simulink model "ForwardKinematic_YuMi"  (R2024a)
(part 8 of 23)

Jacobian_left = [(973764137223015786259973668329660771163465792108934354094153261381447822936595819206046373024901212106219886775732921677418044357043373*sin(q1L))/56784275335594288324165922491250354246378231303696723459491421810987444383859212759858675837012778559434572000489545151057390752235520000 - (89044539378776407626383878029300732391902246482356429453424426540503686155769084630894908573032444807606609378851922454344544769346221*cos(q1L))/28392137667797144162082961245625177123189115651848361729745710905493722191929606379929337918506389279717286000244772575528695376117760000 - (2436553109258773196144549622003023*cos(q6L)*((7514214926474921*cos(q5L)*(((4503599440548691*cos(q4L))/4503599627370496 - (7514214926474921*sin(q4L))/36893488147419103232)*((9007199067919185*sin(q3L)*((46370457884011341126541404977865*cos(q1L))/81129638414606681695789005144064 + (17012367886825063216155529491255*sin(q1L))/162259276829213363391578010288128))/9007199254740992 - cos(q3L)*(cos(q2L)*((1888752292310023*cos(q1L))/18014398509481984 - (5148155107303929*sin(q1L))/9007199254740992) + (7514214926474921*sin(q2L)*((5148155107303929*cos(q1L))/9007199254740992 + (1888752292310023*sin(q1L))/18014398509481984))/36893488147419103232) + (7514214926474921*sin(q3L)*((7514214926474921*cos(q2L)*((5148155107303929*cos(q1L))/9007199254740992 + (1888752292310023*sin(q1L))/18014398509481984))/36893488147419103232 - sin(q2L)*((1888752292310023*cos(q1L))/18014398509481984 - (5148155107303929*sin(q1L))/9007199254740992)))/36893488147419103232) + ((234819211581865*cos(q4L))/1152921504606846976 + (9007199067919185*sin(q4L))/9007199254740992)*((348437586779514700475067630180842053206482623665*cos(q1L))/2993155353253689176481146537402947624255349848014848 + (127834588709863499538908289888301307693646315855*sin(q1L))/5986310706507378352962293074805895248510699696029696 - (67682029681889335677290557259385*cos(q2L)*((5148155107303929*cos(q1L))/9007199254740992 + (1888752292310023*sin(q1L))/18014398509481984))/332306998946228968225951765070086144 + (9007199067919185*sin(q2L)*((1888752292310023*cos(q1L))/18014398509481984 - (5148155107303929*sin(q1L))/9007199254740992))/9007199254740992) + (7514214926474921*cos(q4L)*((9007199067919185*cos(q3L)*((46370457884011341126541404977865*cos(q1L))/81129638414606681695789005144064 + (17012367886825063216155529491255*sin(q1L))/162259276829213363391578010288128))/9007199254740992 + (7514214926474921*cos(q3L)*((7514214926474921*cos(q2L)*((5148155107303929*cos(q1L))/9007199254740992 + (1888752292310023*sin(q1L))/18014398509481984))/36893488147419103232 - sin(q2L)*((1888752292310023*cos(q1L))/18014398509481984 - (5148155107303929*sin(q1L))/9007199254740992)))/36893488147419103232 + sin(q3L)*(cos(q2L)*((1888752292310023*cos(q1L))/18014398509481984 - (5148155107303929*sin(q1L))/9007199254740992) + (7514214926474921*sin(q2L)*((5148155107303929*cos(q1L))/9007199254740992 + (1888752292310023*sin(q1L))/18014398509481984))/36893488147419103232)))/36893488147419103232))/36893488147419103232 + sin(q5L)*(((7514214926474921*cos(q4L))/36893488147419103232 + (4503599440548691*sin(q4L))/4503599627370496)*((9007199067919185*sin(q3L)*((46370457884011341126541404977865*cos(q1L))/81129638414606681695789005144064 + (17012367886825063216155529491255*sin(q1L))/162259276829213363391578010288128))/9007199254740992 - cos(q3L)*(cos(q2L)*((1888752292310023*cos(q1L))/18014398509481984 - (5148155107303929*sin(q1L))/9007199254740992) + (7514214926474921*sin(q2L)*((5148155107303929*cos(q1L))/9007199254740992 + (1888752292310023*sin(q1L))/18014398509481984))/36893488147419103232) + (7514214926474921*sin(q3L)*((7514214926474921*cos(q2L)*((5148155107303929*cos(q1L))/9007199254740992 + (1888752292310023*sin(q1L))/18014398509481984))/36893488147419103232 - sin(q2L)*((1888752292310023*cos(q1L))/18014398509481984 - (5148155107303929*sin(q1L))/9007199254740992)))/36893488147419103232) - ((9007199067919185*cos(q4L))/9007199254740992 - (234819211581865*sin(q4L))/1152921504606846976)*((348437586779514700475067630180842053206482623665*cos(q1L))/2993155353253689176481146537402947624255349848014848 + (127834588709863499538908289888301307693646315855*sin(q1L))/5986310706507378352962293074805895248510699696029696 - (67682029681889335677290557259385*cos(q2L)*((5148155107303929*cos(q1L))/9007199254740992 + (1888752292310023*sin(q1L))/18014398509481984))/332306998946228968225951765070086144 + (9007199067919185*sin(q2L)*((1888752292310023*cos(q1L))/18014398509481984 - (5148155107303929*sin(q1L))/9007199254740992))/9007199254740992) + (7514214926474921*sin(q4L)*((9007199067919185*cos(q3L)*((46370457884011341126541404977865*cos(q1L))/81129638414606681695789005144064 + (17012367886825063216155529491255*sin(q1L))/162259276829213363391578010288128))/9007199254740992 + (7514214926474921*cos(q3L)*((7514214926474921*cos(q2L)*((5148155107303929*cos(q1L))/9007199254740992 + (1888752292310023*sin(q1L))/18014398509481984))/36893488147419103232 - sin(q2L)*((1888752292310023*cos(q1L))/18014398509481984 - (5148155107303929*sin(q1L))/9007199254740992)))/36893488147419103232 + sin(q3L)*(cos(q2L)*((1888752292310023*cos(q1L))/18014398509481984 - (5148155107303929*sin(q1L))/9007199254740992) + (7514214926474921*sin(q2L)*((5148155107303929*cos(q1L))/9007199254740992 + (1888752292310023*sin(q1L))/18014398509481984))/36893488147419103232)))/36893488147419103232) - (9007199067919185*cos(q5L)*((546062636309760713610973115066597791006802105742542518556166375*cos(q1L))/113078212145816597093331040047546785012958969400039613319782796882727665664 + (200339157344278917575443724098432450908090682630030995291449625*sin(q1L))/226156424291633194186662080095093570025917938800079226639565593765455331328 - (81129635049124235038645691064225*cos(q3L)*((46370457884011341126541404977865*cos(q1L))/81129638414606681695789005144064 + (17012367886825063216155529491255*sin(q1L))/162259276829213363391578010288128))/81129638414606681695789005144064 + (2115063383689692319117831580025*sin(q3L)*((46370457884011341126541404977865*cos(q1L))/81129638414606681695789005144064 + (17012367886825063216155529491255*sin(q1L))/162259276829213363391578010288128))/10384593717069655257060992658440192 - (234819211581865*cos(q3L)*(cos(q2L)*((1888752292310023*cos(q1L))/18014398509481984 - (5148155107303929*sin(q1L))/9007199254740992) + (7514214926474921*sin(q2L)*((5148155107303929*cos(q1L))/9007199254740992 + (1888752292310023*sin(q1L))/18014398509481984))/36893488147419103232))/1152921504606846976 - (67682029681889335677290557259385*cos(q3L)*((7514214926474921*cos(q2L)*((5148155107303929*cos(q1L))/9007199254740992 + (1888752292310023*sin(q1L))/18014398509481984))/36893488147419103232 - sin(q2L)*((1888752292310023*cos(q1L))/18014398509481984 - (5148155107303929*sin(q1L))/9007199254740992)))/332306998946228968225951765070086144 - (9007199067919185*sin(q3L)*(cos(q2L)*((1888752292310023*cos(q1L))/18014398509481984 - (5148155107303929*sin(q1L))/9007199254740992) + (7514214926474921*sin(q2L)*((5148155107303929*cos(q1L))/9007199254740992 + (1888752292310023*sin(q1L))/18014398509481984))/36893488147419103232))/9007199254740992 + (1764482024691522628700660907665*sin(q3L)*((7514214926474921*cos(q2L)*((5148155107303929*cos(q1L))/9007199254740992 + (1888752292310023*sin(q1L))/18014398509481984))/36893488147419103232 - sin(q2L)*((1888752292310023*cos(q1L))/18014398509481984 - (5148155107303929*sin(q1L))/9007199254740992)))/42535295865117307932921825928971026432 - (106069577339469832923929692356850887620017617375*cos(q2L)*((5148155107303929*cos(q1L))/9007199254740992 + (1888752292310023*sin(q1L))/18014398509481984))/12554203470773361527671578846415332832204710888928069025792 + (14115856197532180673579726082375*sin(q2L)*((1888752292310023*cos(q1L))/18014398509481984 - (5148155107303929*sin(q1L))/9007199254740992))/340282366920938463463374607431768211456))/9007199254740992))/332306998946228968225951765070086144000 - (81222263116692158804177042061221826384594597321566869716687*((4503599440548691*cos(q4L))/4503599627370496 - (7514214926474921*sin(q4L))/36893488147419103232)*((9007199067919185*sin(q3L)*((46370457884011341126541404977865*cos(q1L))/81129638414606681695789005144064 + (17012367886825063216155529491255*sin(q1L))/162259276829213363391578010288128))/9007199254740992 - cos(q3L)*(cos(q2L)*((1888752292310023*cos(q1L))/18014398509481984 - (5148155107303929*sin(q1L))/9007199254740992) + (7514214926474921*sin(q2L)*((5148155107303929*cos(q1L))/9007199254740992 + (1888752292310023*sin(q1L))/18014398509481984))/36893488147419103232) + (7514214926474921*sin(q3L)*((7514214926474921*cos(q2L)*((5148155107303929*cos(q1L))/9007199254740992 + (1888752292310023*sin(q1L))/18014398509481984))/36893488147419103232 - sin(q2L)*((1888752292310023*cos(q1L))/18014398509481984 - (5148155107303929*sin(q1L))/9007199254740992)))/36893488147419103232))/306499108173177771671669405430061836723747824436720435200000 - (81*((7514214926474921*cos(q4L))/36893488147419103232 + (4503599440548691*sin(q4L))/4503599627370496)*((9007199067919185*sin(q3L)*((46370457884011341126541404977865*cos(q1L))/81129638414606681695789005144064 + (17012367886825063216155529491255*sin(q1L))/162259276829213363391578010288128))/9007199254740992 - cos(q3L)*(cos(q2L)*((1888752292310023*cos(q1L))/18014398509481984 - (5148155107303929*sin(q1L))/9007199254740992) + (7514214926474921*sin(q2L)*((5148155107303929*cos(q1L))/9007199254740992 + (1888752292310023*sin(q1L))/18014398509481984))/36893488147419103232) + (7514214926474921*sin(q3L)*((7514214926474921*cos(q2L)*((5148155107303929*cos(q1L))/9007199254740992 + (1888752292310023*sin(q1L))/18014398509481984))/36893488147419103232 - sin(q2L)*((1888752292310023*cos(q1L))/18014398509481984 - (5148155107303929*sin(q1L))/9007199254740992)))/36893488147419103232))/2000 - (27*cos(q6L)*(cos(q5L)*(((7514214926474921*cos(q4L))/36893488147419103232 + (4503599440548691*sin(q4L))/4503599627370496)*((9007199067919185*sin(q3L)*((46370457884011341126541404977865*cos(q1L))/81129638414606681695789005144064 + (17012367886825063216155529491255*sin(q1L))/162259276829213363391578010288128))/9007199254740992 - cos(q3L)*(cos(q2L)*((1888752292310023*cos(q1L))/18014398509481984 - (5148155107303929*sin(q1L))/9007199254740992) + (7514214926474921*sin(q2L)*((5148155107303929*cos(q1L))/9007199254740992 + (1888752292310023*sin(q1L))/18014398509481984))/36893488147419103232) + (7514214926474921*sin(q3L)*((7514214926474921*cos(q2L)*((5148155107303929*cos(q1L))/9007199254740992 + (1888752292310023*sin(q1L))/18014398509481984))/36893488147419103232 - sin(q2L)*((1888752292310023*cos(q1L))/18014398509481984 - (5148155107303929*sin(q1L))/9007199254740992)))/36893488147419103232) - ((9007199067919185*cos(q4L))/9007199254740992 - (234819211581865*sin(q4L))/1152921504606846976)*((348437586779514700475067630180842053206482623665*cos(q1L))/2993155353253689176481146537402947624255349848014848 + (127834588709863499538908289888301307693646315855*sin(q1L))/5986310706507378352962293074805895248510699696029696 - (67682029681889335677290557259385*cos(q2L)*((5148155107303929*cos(q1L))/9007199254740992 + (1888752292310023*sin(q1L))/18014398509481984))/332306998946228968225951765070086144 + (9007199067919185*sin(q2L)*((1888752292310023*cos(q1L))/18014398509481984 - (5148155107303929*sin(q1L))/9007199254740992))/9007199254740992) + (7514214926474921*sin(q4L)*((9007199067919185*cos(q3L)*((46370457884011341126541404977865*cos(q1L))/81129638414606681695789005144064 + (17012367886825063216155529491255*sin(q1L))/162259276829213363391578010288128))/9007199254740992 + (7514214926474921*cos(q3L)*((7514214926474921*cos(q2L)*((5148155107303929*cos(q1L))/9007199254740992 + (1888752292310023*sin(q1L))/18014398509481984))/36893488147419103232 - sin(q2L)*((1888752292310023*cos(q1L))/18014398509481984 - (5148155107303929*sin(q1L))/9007199254740992)))/36893488147419103232 + sin(q3L)*(cos(q2L)*((1888752292310023*cos(q1L))/18014398509481984 - (5148155107303929*sin(q1L))/9007199254740992) + (7514214926474921*sin(q2L)*((5148155107303929*cos(q1L))/9007199254740992 + (1888752292310023*sin(q1L))/18014398509481984))/36893488147419103232)))/36893488147419103232) - (7514214926474921*sin(q5L)*(((4503599440548691*cos(q4L))/4503599627370496 - (7514214926474921*sin(q4L))/36893488147419103232)*((9007199067919185*sin(q3L)*((46370457884011341126541404977865*cos(q1L))/81129638414606681695789005144064 + (17012367886825063216155529491255*sin(q1L))/162259276829213363391578010288128))/9007199254740992 - cos(q3L)*(cos(q2L)*((1888752292310023*cos(q1L))/18014398509481984 - (5148155107303929*sin(q1L))/9007199254740992) + (7514214926474921*sin(q2L)*((5148155107303929*cos(q1L))/9007199254740992 + (1888752292310023*sin(q1L))/18014398509481984))/36893488147419103232) + (7514214926474921*sin(q3L)*((7514214926474921*cos(q2L)*((5148155107303929*cos(q1L))/9007199254740992 + (1888752292310023*sin(q1L))/18014398509481984))/36893488147419103232 - sin(q2L)*((1888752292310023*cos(q1L))/18014398509481984 - (5148155107303929*sin(q1L))/9007199254740992)))/36893488147419103232) + ((234819211581865*cos(q4L))/1152921504606846976 + (9007199067919185*sin(q4L))/9007199254740992)*((348437586779514700475067630180842053206482623665*cos(q1L))/2993155353253689176481146537402947624255349848014848 + (127834588709863499538908289888301307693646315855*sin(q1L))/5986310706507378352962293074805895248510699696029696 - (67682029681889335677290557259385*cos(q2L)*((5148155107303929*cos(q1L))/9007199254740992 + (1888752292310023*sin(q1L))/18014398509481984))/332306998946228968225951765070086144 + (9007199067919185*sin(q2L)*((1888752292310023*cos(q1L))/18014398509481984 - (5148155107303929*sin(q1L))/9007199254740992))/9007199254740992) + (7514214926474921*cos(q4L)*((9007199067919185*cos(q3L)*((46370457884011341126541404977865*cos(q1L))/81129638414606681695789005144064 + (17012367886825063216155529491255*sin(q1L))/162259276829213363391578010288128))/9007199254740992 + (7514214926474921*cos(q3L)*((7514214926474921*cos(q2L)*((5148155107303929*cos(q1L))/9007199254740992 + (1888752292310023*sin(q1L))/18014398509481984))/36893488147419103232 - sin(q2L)*((1888752292310023*cos(q1L))/18014398509481984 - (5148155107303929*sin(q1L))/9007199254740992)))/36893488147419103232 + sin(q3L)*(cos(q2L)*((1888752292310023*cos(q1L))/18014398509481984 - (5148155107303929*sin(q1L))/9007199254740992) + (7514214926474921*sin(q2L)*((5148155107303929*cos(q1L))/9007199254740992 + (1888752292310023*sin(q1L))/18014398509481984))/36893488147419103232)))/36893488147419103232))/36893488147419103232 + (9007199067919185*sin(q5L)*((546062636309760713610973115066597791006802105742542518556166375*cos(q1L))/113078212145816597093331040047546785012958969400039613319782796882727665664 + (200339157344278917575443724098432450908090682630030995291449625*sin(q1L))/226156424291633194186662080095093570025917938800079226639565593765455331328 - (81129635049124235038645691064225*cos(q3L)*((46370457884011341126541404977865*cos(q1L))/81129638414606681695789005144064 + (17012367886825063216155529491255*sin(q1L))/162259276829213363391578010288128))/81129638414606681695789005144064 + (2115063383689692319117831580025*sin(q3L)*((46370457884011341126541404977865*cos(q1L))/81129638414606681695789005144064 + (17012367886825063216155529491255*sin(q1L))/162259276829213363391578010288128))/10384593717069655257060992658440192 - (234819211581865*cos(q3L)*(cos(q2L)*((1888752292310023*cos(q1L))/18014398509481984 - (5148155107303929*sin(q1L))/9007199254740992) + (7514214926474921*sin(q2L)*((5148155107303929*cos(q1L))/9007199254740992 + (1888752292310023*sin(q1L))/18014398509481984))/36893488147419103232))/1152921504606846976 - (67682029681889335677290557259385*cos(q3L)*((7514214926474921*cos(q2L)*((5148155107303929*cos(q1L))/9007199254740992 + (1888752292310023*sin(q1L))/18014398509481984))/36893488147419103232 - sin(q2L)*((1888752292310023*cos(q1L))/18014398509481984 - (5148155107303929*sin(q1L))/9007199254740992)))/332306998946228968225951765070086144 - (9007199067919185*sin(q3L)*(cos(q2L)*((1888752292310023*cos(q1L))/18014398509481984 - (5148155107303929*sin(q1L))/9007199254740992) + (7514214926474921*sin(q2L)*((5148155107303929*cos(q1L))/9007199254740992 + (1888752292310023*sin(q1L))/18014398509481984))/36893488147419103232))/9007199254740992 + (1764482024691522628700660907665*sin(q3L)*((7514214926474921*cos(q2L)*((5148155107303929*cos(q1L))/9007199254740992 + (1888752292310023*sin(q1L))/18014398509481984))/36893488147419103232 - sin(q2L)*((1888752292310023*cos(q1L))/18014398509481984 - (5148155107303929*sin(q1L))/9007199254740992)))/42535295865117307932921825928971026432 - (106069577339469832923929692356850887620017617375*cos(q2L)*((5148155107303929*cos(q1L))/9007199254740992 + (1888752292310023*sin(q1L))/18014398509481984))/12554203470773361527671578846415332832204710888928069025792 + (14115856197532180673579726082375*sin(q2L)*((1888752292310023*cos(q1L))/18014398509481984 - (5148155107303929*sin(q1L))/9007199254740992))/340282366920938463463374607431768211456))/9007199254740992))/1000 - (202883803014822867*sin(q6L)*((7514214926474921*cos(q5L)*(((4503599440548691*cos(q4L))/4503599627370496 - (7514214926474921*sin(q4L))/36893488147419103232)*((9007199067919185*sin(q3L)*((46370457884011341126541404977865*cos(q1L))/81129638414606681695789005144064 + (17012367886825063216155529491255*sin(q1L))/162259276829213363391578010288128))/9007199254740992 - cos(q3L)*(cos(q2L)*((1888752292310023*cos(q1L))/18014398509481984 - (5148155107303929*sin(q1L))/9007199254740992) + (7514214926474921*sin(q2L)*((5148155107303929*cos(q1L))/9007199254740992 + (1888752292310023*sin(q1L))/18014398509481984))/36893488147419103232) + (7514214926474921*sin(q3L)*((7514214926474921*cos(q2L)*((5148155107303929*cos(q1L))/9007199254740992 + (1888752292310023*sin(q1L))/18014398509481984))/36893488147419103232 - sin(q2L)*((1888752292310023*cos(q1L))/18014398509481984 - (5148155107303929*sin(q1L))/9007199254740992)))/36893488147419103232) + ((234819211581865*cos(q4L))/1152921504606846976 + (9007199067919185*sin(q4L))/9007199254740992)*((348437586779514700475067630180842053206482623665*cos(q1L))/2993155353253689176481146537402947624255349848014848 + (127834588709863499538908289888301307693646315855*sin(q1L))/5986310706507378352962293074805895248510699696029696 - (67682029681889335677290557259385*cos(q2L)*((5148155107303929*cos(q1L))/9007199254740992 + (1888752292310023*sin(q1L))/18014398509481984))/332306998946228968225951765070086144 + (9007199067919185*sin(q2L)*((1888752292310023*cos(q1L))/18014398509481984 - (5148155107303929*sin(q1L))/9007199254740992))/9007199254740992) + (7514214926474921*cos(q4L)*((9007199067919185*cos(q3L)*((46370457884011341126541404977865*cos(q1L))/81129638414606681695789005144064 + (17012367886825063216155529491255*sin(q1L))/162259276829213363391578010288128))/9007199254740992 + (7514214926474921*cos(q3L)*((7514214926474921*cos(q2L)*((5148155107303929*cos(q1L))/9007199254740992 + (1888752292310023*sin(q1L))/18014398509481984))/36893488147419103232 - sin(q2L)*((1888752292310023*cos(q1L))/18014398509481984 - (5148155107303929*sin(q1L))/9007199254740992)))/36893488147419103232 + sin(q3L)*(cos(q2L)*((1888752292310023*cos(q1L))/18014398509481984 - (5148155107303929*sin(q1L))/9007199254740992) + (7514214926474921*sin(q2L)*((5148155107303929*cos(q1L))/9007199254740992 + (1888752292310023*sin(q1L))/18014398509481984))/36893488147419103232)))/36893488147419103232))/36893488147419103232 + sin(q5L)*(((7514214926474921*cos(q4L))/36893488147419103232 + (4503599440548691*sin(q4L))/4503599627370496)*((9007199067919185*sin(q3L)*((46370457884011341126541404977865*cos(q1L))/81129638414606681695789005144064 + (17012367886825063216155529491255*sin(q1L))/162259276829213363391578010288128))/9007199254740992 - cos(q3L)*(cos(q2L)*((1888752292310023*cos(q1L))/18014398509481984 - (5148155107303929*sin(q1L))/9007199254740992) + (7514214926474921*sin(q2L)*((5148155107303929*cos(q1L))/9007199254740992 + (1888752292310023*sin(q1L))/18014398509481984))/36893488147419103232) + (7514214926474921*sin(q3L)*((7514214926474921*cos(q2L)*((5148155107303929*cos(q1L))/9007199254740992 + (1888752292310023*sin(q1L))/18014398509481984))/36893488147419103232 - sin(q2L)*((1888752292310023*cos(q1L))/18014398509481984 - (5148155107303929*sin(q1L))/9007199254740992)))/36893488147419103232) - ((9007199067919185*cos(q4L))/9007199254740992 - (234819211581865*sin(q4L))/1152921504606846976)*((348437586779514700475067630180842053206482623665*cos(q1L))/2993155353253689176481146537402947624255349848014848 + (127834588709863499538908289888301307693646315855*sin(q1L))/5986310706507378352962293074805895248510699696029696 - (67682029681889335677290557259385*cos(q2L)*((5148155107303929*cos(q1L))/9007199254740992 + (1888752292310023*sin(q1L))/18014398509481984))/332306998946228968225951765070086144 + (9007199067919185*sin(q2L)*((1888752292310023*cos(q1L))/18014398509481984 - (5148155107303929*sin(q1L))/9007199254740992))/9007199254740992) + (7514214926474921*sin(q4L)*((9007199067919185*cos(q3L)*((46370457884011341126541404977865*cos(q1L))/81129638414606681695789005144064 + (17012367886825063216155529491255*sin(q1L))/162259276829213363391578010288128))/9007199254740992 + (7514214926474921*cos(q3L)*((7514214926474921*cos(q2L)*((5148155107303929*cos(q1L))/9007199254740992 + (1888752292310023*sin(q1L))/18014398509481984))/36893488147419103232 - sin(q2L)*((1888752292310023*cos(q1L))/18014398509481984 - (5148155107303929*sin(q1L))/9007199254740992)))/36893488147419103232 + sin(q3L)*(cos(q2L)*((1888752292310023*cos(q1L))/18014398509481984 - (5148155107303929*sin(q1L))/9007199254740992) + (7514214926474921*sin(q2L)*((5148155107303929*cos(q1L))/9007199254740992 + (1888752292310023*sin(q1L))/18014398509481984))/36893488147419103232)))/36893488147419103232) - (9007199067919185*cos(q5L)*((546062636309760713610973115066597791006802105742542518556166375*cos(q1L))/113078212145816597093331040047546785012958969400039613319782796882727665664 + (200339157344278917575443724098432450908090682630030995291449625*sin(q1L))/226156424291633194186662080095093570025917938800079226639565593765455331328 - (81129635049124235038645691064225*cos(q3L)*((46370457884011341126541404977865*cos(q1L))/81129638414606681695789005144064 + (17012367886825063216155529491255*sin(q1L))/162259276829213363391578010288128))/81129638414606681695789005144064 + (2115063383689692319117831580025*sin(q3L)*((46370457884011341126541404977865*cos(q1L))/81129638414606681695789005144064 + (17012367886825063216155529491255*sin(q1L))/162259276829213363391578010288128))/10384593717069655257060992658440192 - (234819211581865*cos(q3L)*(cos(q2L)*((1888752292310023*cos(q1L))/18014398509481984 - (5148155107303929*sin(q1L))/9007199254740992) + (7514214926474921*sin(q2L)*((5148155107303929*cos(q1L))/9007199254740992 + (1888752292310023*sin(q1L))/18014398509481984))/36893488147419103232))/1152921504606846976 - (67682029681889335677290557259385*cos(q3L)*((7514214926474921*cos(q2L)*((5148155107303929*cos(q1L))/9007199254740992 + (1888752292310023*sin(q1L))/18014398509481984))/36893488147419103232 - sin(q2L)*((1888752292310023*cos(q1L))/18014398509481984 - (5148155107303929*sin(q1L))/9007199254740992)))/332306998946228968225951765070086144 - (9007199067919185*sin(q3L)*(cos(q2L)*((1888752292310023*cos(q1L))/18014398509481984 - (5148155107303929*sin(q1L))/9007199254740992) + (7514214926474921*sin(q2L)*((5148155107303929*cos(q1L))/9007199254740992 + (1888752292310023*sin(q1L))/18014398509481984))/36893488147419103232))/9007199254740992 + (1764482024691522628700660907665*sin(q3L)*((7514214926474921*cos(q2L)*((5148155107303929*cos(q1L))/9007199254740992 + (1888752292310023*sin(q1L))/18014398509481984))/36893488147419103232 - sin(q2L)*((1888752292310023*cos(q1L))/18014398509481984 - (5148155107303929*sin(q1L))/9007199254740992)))/42535295865117307932921825928971026432 - (106069577339469832923929692356850887620017617375*cos(q2L)*((5148155107303929*cos(q1L))/9007199254740992 + (1888752292310023*sin(q1L))/18014398509481984))/12554203470773361527671578846415332832204710888928069025792 + (14115856197532180673579726082375*sin(q2L)*((1888752292310023*cos(q1L))/18014398509481984 - (5148155107303929*sin(q1L))/9007199254740992))/340282366920938463463374607431768211456))/9007199254740992))/36893488147419103232000 + (324259171862923063*sin(q6L)*(cos(q5L)*(((7514214926474921*cos(q4L))/36893488147419103232 + (4503599440548691*sin(q4L))/4503599627370496)*((9007199067919185*sin(q3L)*((46370457884011341126541404977865*cos(q1L))/81129638414606681695789005144064 + (17012367886825063216155529491255*sin(q1L))/162259276829213363391578010288128))/9007199254740992 - cos(q3L)*(cos(q2L)*((1888752292310023*cos(q1L))/18014398509481984 - (5148155107303929*sin(q1L))/9007199254740992) + (7514214926474921*sin(q2L)*((5148155107303929*cos(q1L))/9007199254740992 + (1888752292310023*sin(q1L))/18014398509481984))/36893488147419103232) + (7514214926474921*sin(q3L)*((7514214926474921*cos(q2L)*((5148155107303929*cos(q1L))/9007199254740992 + (1888752292310023*sin(q1L))/18014398509481984))/36893488147419103232 - sin(q2L)*((1888752292310023*cos(q1L))/18014398509481984 - (5148155107303929*sin(q1L))/9007199254740992)))/36893488147419103232) - ((9007199067919185*cos(q4L))/9007199254740992 - (234819211581865*sin(q4L))/1152921504606846976)*((348437586779514700475067630180842053206482623665*cos(q1L))/2993155353253689176481146537402947624255349848014848 + (127834588709863499538908289888301307693646315855*sin(q1L))/5986310706507378352962293074805895248510699696029696 - (67682029681889335677290557259385*cos(q2L)*((5148155107303929*cos(q1L))/9007199254740992 + (1888752292310023*sin(q1L))/18014398509481984))/332306998946228968225951765070086144 + (9007199067919185*sin(q2L)*((1888752292310023*cos(q1L))/18014398509481984 - (5148155107303929*sin(q1L))/9007199254740992))/9007199254740992) + (7514214926474921*sin(q4L)*((9007199067919185*cos(q3L)*((46370457884011341126541404977865*cos(q1L))/81129638414606681695789005144064 + (17012367886825063216155529491255*sin(q1L))/162259276829213363391578010288128))/9007199254740992 + (7514214926474921*cos(q3L)*((7514214926474921*cos(q2L)*((5148155107303929*cos(q1L))/9007199254740992 + (1888752292310023*sin(q1L))/18014398509481984))/36893488147419103232 - sin(q2L)*((1888752292310023*cos(q1L))/18014398509481984 - (5148155107303929*sin(q1L))/9007199254740992)))/36893488147419103232 + sin(q3L)*(cos(q2L)*((1888752292310023*cos(q1L))/18014398509481984 - (5148155107303929*sin(q1L))/9007199254740992) + (7514214926474921*sin(q2L)*((5148155107303929*cos(q1L))/9007199254740992 + (1888752292310023*sin(q1L))/18014398509481984))/36893488147419103232)))/36893488147419103232) - (7514214926474921*sin(q5L)*(((4503599440548691*cos(q4L))/4503599627370496 - (7514214926474921*sin(q4L))/36893488147419103232)*((9007199067919185*sin(q3L)*((46370457884011341126541404977865*cos(q1L))/81129638414606681695789005144064 + (17012367886825063216155529491255*sin(q1L))/162259276829213363391578010288128))/9007199254740992 - cos(q3L)*(cos(q2L)*((1888752292310023*cos(q1L))/18014398509481984 - (5148155107303929*sin(q1L))/9007199254740992) + (7514214926474921*sin(q2L)*((5148155107303929*cos(q1L))/9007199254740992 + (1888752292310023*sin(q1L))/18014398509481984))/36893488147419103232) + (7514214926474921*sin(q3L)*((7514214926474921*cos(q2L)*((5148155107303929*cos(q1L))/9007199254740992 + (1888752292310023*sin(q1L))/18014398509481984))/36893488147419103232 - sin(q2L)*((1888752292310023*cos(q1L))/18014398509481984 - (5148155107303929*sin(q1L))/9007199254740992)))/36893488147419103232) + ((234819211581865*cos(q4L))/1152921504606846976 + (9007199067919185*sin(q4L))/9007199254740992)*((348437586779514700475067630180842053206482623665*cos(q1L))/2993155353253689176481146537402947624255349848014848 + (127834588709863499538908289888301307693646315855*sin(q1L))/5986310706507378352962293074805895248510699696029696 - (67682029681889335677290557259385*cos(q2L)*((5148155107303929*cos(q1L))/9007199254740992 + (1888752292310023*sin(q1L))/18014398509481984))/332306998946228968225951765070086144 + (9007199067919185*sin(q2L)*((1888752292310023*cos(q1L))/18014398509481984 - (5148155107303929*sin(q1L))/9007199254740992))/9007199254740992) + (7514214926474921*cos(q4L)*((9007199067919185*cos(q3L)*((46370457884011341126541404977865*cos(q1L))/81129638414606681695789005144064 + (17012367886825063216155529491255*sin(q1L))/162259276829213363391578010288128))/9007199254740992 + (7514214926474921*cos(q3L)*((7514214926474921*cos(q2L)*((5148155107303929*cos(q1L))/9007199254740992 + (1888752292310023*sin(q1L))/18014398509481984))/36893488147419103232 - sin(q2L)*((1888752292310023*cos(q1L))/18014398509481984 - (5148155107303929*sin(q1L))/9007199254740992)))/36893488147419103232 + sin(q3L)*(cos(q2L)*((1888752292310023*cos(q1L))/18014398509481984 - (5148155107303929*sin(q1L))/9007199254740992) + (7514214926474921*sin(q2L)*((5148155107303929*cos(q1L))/9007199254740992 + (1888752292310023*sin(q1L))/18014398509481984))/36893488147419103232)))/36893488147419103232))/36893488147419103232 + (9007199067919185*sin(q5L)*((546062636309760713610973115066597791006802105742542518556166375*cos(q1L))/113078212145816597093331040047546785012958969400039613319782796882727665664 + (200339157344278917575443724098432450908090682630030995291449625*sin(q1L))/226156424291633194186662080095093570025917938800079226639565593765455331328 - (81129635049124235038645691064225*cos(q3L)*((46370457884011341126541404977865*cos(q1L))/81129638414606681695789005144064 + (17012367886825063216155529491255*sin(q1L))/162259276829213363391578010288128))/81129638414606681695789005144064 + (2115063383689692319117831580025*sin(q3L)*((46370457884011341126541404977865*cos(q1L))/81129638414606681695789005144064 + (17012367886825063216155529491255*sin(q1L))/162259276829213363391578010288128))/10384593717069655257060992658440192 - (234819211581865*cos(q3L)*(cos(q2L)*((1888752292310023*cos(q1L))/18014398509481984 - (5148155107303929*sin(q1L))/9007199254740992) + (7514214926474921*sin(q2L)*((5148155107303929*cos(q1L))/9007199254740992 + (1888752292310023*sin(q1L))/18014398509481984))/36893488147419103232))/1152921504606846976 - (67682029681889335677290557259385*cos(q3L)*((7514214926474921*cos(q2L)*((5148155107303929*cos(q1L))/9007199254740992 + (1888752292310023*sin(q1L))/18014398509481984))/36893488147419103232 - sin(q2L)*((1888752292310023*cos(q1L))/18014398509481984 - (5148155107303929*sin(q1L))/9007199254740992)))/332306998946228968225951765070086144 - (9007199067919185*sin(q3L)*(cos(q2L)*((1888752292310023*cos(q1L))/18014398509481984 - (5148155107303929*sin(q1L))/9007199254740992) + (7514214926474921*sin(q2L)*((5148155107303929*cos(q1L))/9007199254740992 + (1888752292310023*sin(q1L))/18014398509481984))/36893488147419103232))/9007199254740992 + (1764482024691522628700660907665*sin(q3L)*((7514214926474921*cos(q2L)*((5148155107303929*cos(q1L))/9007199254740992 + (1888752292310023*sin(q1L))/18014398509481984))/36893488147419103232 - sin(q2L)*((1888752292310023*cos(q1L))/18014398509481984 - (5148155107303929*sin(q1L))/9007199254740992)))/42535295865117307932921825928971026432 - (106069577339469832923929692356850887620017617375*cos(q2L)*((5148155107303929*cos(q1L))/9007199254740992 + (1888752292310023*sin(q1L))/18014398509481984))/12554203470773361527671578846415332832204710888928069025792 + (14115856197532180673579726082375*sin(q2L)*((1888752292310023*cos(q1L))/18014398509481984 - (5148155107303929*sin(q1L))/9007199254740992))/340282366920938463463374607431768211456))/9007199254740992))/9007199254740992000 + (83301539375654672537075965313343183841442266989297270401707771044036658496661398777306991*cos(q3L)*((46370457884011341126541404977865*cos(q1L))/81129638414606681695789005144064 + (17012367886825063216155529491255*sin(q1L))/162259276829213363391578010288128))/4074071952668972172536891376818756322102936787331872501272280898708762599526673412366794752000 - (109198173955282063961996941994332957526645881091499469714283881779231664456243735535448036415347*sin(q3L)*((46370457884011341126541404977865*cos(q1L))/81129638414606681695789005144064 + (17012367886825063216155529491255*sin(q1L))/162259276829213363391578010288128))/2607406049708142190423610481164004046145879543892398400814259775173608063697070983914748641280000 + (81*((9007199067919185*cos(q4L))/9007199254740992 - (234819211581865*sin(q4L))/1152921504606846976)*((348437586779514700475067630180842053206482623665*cos(q1L))/2993155353253689176481146537402947624255349848014848 + (127834588709863499538908289888301307693646315855*sin(q1L))/5986310706507378352962293074805895248510699696029696 - (67682029681889335677290557259385*cos(q2L)*((5148155107303929*cos(q1L))/9007199254740992 + (1888752292310023*sin(q1L))/18014398509481984))/332306998946228968225951765070086144 + (9007199067919185*sin(q2L)*((1888752292310023*cos(q1L))/18014398509481984 - (5148155107303929*sin(q1L))/9007199254740992))/9007199254740992))/2000 - (81222263116692158804177042061221826384594597321566869716687*((234819211581865*cos(q4L))/1152921504606846976 + (9007199067919185*sin(q4L))/9007199254740992)*((348437586779514700475067630180842053206482623665*cos(q1L))/2993155353253689176481146537402947624255349848014848 + (127834588709863499538908289888301307693646315855*sin(q1L))/5986310706507378352962293074805895248510699696029696 - (67682029681889335677290557259385*cos(q2L)*((5148155107303929*cos(q1L))/9007199254740992 + (1888752292310023*sin(q1L))/18014398509481984))/332306998946228968225951765070086144 + (9007199067919185*sin(q2L)*((1888752292310023*cos(q1L))/18014398509481984 - (5148155107303929*sin(q1L))/9007199254740992))/9007199254740992))/306499108173177771671669405430061836723747824436720435200000 + (60617164743372705924380750591060836759586313939367162716784907429017787816377231*cos(q3L)*(cos(q2L)*((1888752292310023*cos(q1L))/18014398509481984 - (5148155107303929*sin(q1L))/9007199254740992) + (7514214926474921*sin(q2L)*((5148155107303929*cos(q1L))/9007199254740992 + (1888752292310023*sin(q1L))/18014398509481984))/36893488147419103232))/1447401115466452442794637312608598848165874808320507050493219800098914120499200000 + (347469655025336708709976918716104493695816557877713443586884917071777956519687017125887603*cos(q3L)*((7514214926474921*cos(q2L)*((5148155107303929*cos(q1L))/9007199254740992 + (1888752292310023*sin(q1L))/18014398509481984))/36893488147419103232 - sin(q2L)*((1888752292310023*cos(q1L))/18014398509481984 - (5148155107303929*sin(q1L))/9007199254740992)))/83436993590660550093555535397248129476668145404556748826056312805555458038306271485271956520960000 + (712008244765680093343103025701132101054572137019*cos(q5L)*(((4503599440548691*cos(q4L))/4503599627370496 - (7514214926474921*sin(q4L))/36893488147419103232)*((9007199067919185*sin(q3L)*((46370457884011341126541404977865*cos(q1L))/81129638414606681695789005144064 + (17012367886825063216155529491255*sin(q1L))/162259276829213363391578010288128))/9007199254740992 - cos(q3L)*(cos(q2L)*((1888752292310023*cos(q1L))/18014398509481984 - (5148155107303929*sin(q1L))/9007199254740992) + (7514214926474921*sin(q2L)*((5148155107303929*cos(q1L))/9007199254740992 + (1888752292310023*sin(q1L))/18014398509481984))/36893488147419103232) + (7514214926474921*sin(q3L)*((7514214926474921*cos(q2L)*((5148155107303929*cos(q1L))/9007199254740992 + (1888752292310023*sin(q1L))/18014398509481984))/36893488147419103232 - sin(q2L)*((1888752292310023*cos(q1L))/18014398509481984 - (5148155107303929*sin(q1L))/9007199254740992)))/36893488147419103232) + ((234819211581865*cos(q4L))/1152921504606846976 + (9007199067919185*sin(q4L))/9007199254740992)*((348437586779514700475067630180842053206482623665*cos(q1L))/2993155353253689176481146537402947624255349848014848 + (127834588709863499538908289888301307693646315855*sin(q1L))/5986310706507378352962293074805895248510699696029696 - (67682029681889335677290557259385*cos(q2L)*((5148155107303929*cos(q1L))/9007199254740992 + (1888752292310023*sin(q1L))/18014398509481984))/332306998946228968225951765070086144 + (9007199067919185*sin(q2L)*((1888752292310023*cos(q1L))/18014398509481984 - (5148155107303929*sin(q1L))/9007199254740992))/9007199254740992) + (7514214926474921*cos(q4L)*((9007199067919185*cos(q3L)*((46370457884011341126541404977865*cos(q1L))/81129638414606681695789005144064 + (17012367886825063216155529491255*sin(q1L))/162259276829213363391578010288128))/9007199254740992 + (7514214926474921*cos(q3L)*((7514214926474921*cos(q2L)*((5148155107303929*cos(q1L))/9007199254740992 + (1888752292310023*sin(q1L))/18014398509481984))/36893488147419103232 - sin(q2L)*((1888752292310023*cos(q1L))/18014398509481984 - (5148155107303929*sin(q1L))/9007199254740992)))/36893488147419103232 + sin(q3L)*(cos(q2L)*((1888752292310023*cos(q1L))/18014398509481984 - (5148155107303929*sin(q1L))/9007199254740992) + (7514214926474921*sin(q2L)*((5148155107303929*cos(q1L))/9007199254740992 + (1888752292310023*sin(q1L))/18014398509481984))/36893488147419103232)))/36893488147419103232))/2451992865385422173373355243440494693789982595493763481600 + (46241644459901303158631016767207157814229090534989303509431886332469146043*sin(q3L)*(cos(q2L)*((1888752292310023*cos(q1L))/18014398509481984 - (5148155107303929*sin(q1L))/9007199254740992) + (7514214926474921*sin(q2L)*((5148155107303929*cos(q1L))/9007199254740992 + (1888752292310023*sin(q1L))/18014398509481984))/36893488147419103232))/2261564242916331941866620800950935700259179388000792266395655937654553313280000 - (455490404115240510935077772268745492204390157443214084883134054419271951750419293234291596923751*sin(q3L)*((7514214926474921*cos(q2L)*((5148155107303929*cos(q1L))/9007199254740992 + (1888752292310023*sin(q1L))/18014398509481984))/36893488147419103232 - sin(q2L)*((1888752292310023*cos(q1L))/18014398509481984 - (5148155107303929*sin(q1L))/9007199254740992)))/53399675898022752059875542654238802865067613058916319248676040195555493144516013750574052173414400000 - (202883803014822867*sin(q5L)*(((4503599440548691*cos(q4L))/4503599627370496 - (7514214926474921*sin(q4L))/36893488147419103232)*((9007199067919185*sin(q3L)*((46370457884011341126541404977865*cos(q1L))/81129638414606681695789005144064 + (17012367886825063216155529491255*sin(q1L))/162259276829213363391578010288128))/9007199254740992 - cos(q3L)*(cos(q2L)*((1888752292310023*cos(q1L))/18014398509481984 - (5148155107303929*sin(q1L))/9007199254740992) + (7514214926474921*sin(q2L)*((5148155107303929*cos(q1L))/9007199254740992 + (1888752292310023*sin(q1L))/18014398509481984))/36893488147419103232) + (7514214926474921*sin(q3L)*((7514214926474921*cos(q2L)*((5148155107303929*cos(q1L))/9007199254740992 + (1888752292310023*sin(q1L))/18014398509481984))/36893488147419103232 - sin(q2L)*((1888752292310023*cos(q1L))/18014398509481984 - (5148155107303929*sin(q1L))/9007199254740992)))/36893488147419103232) + ((234819211581865*cos(q4L))/1152921504606846976 + (9007199067919185*sin(q4L))/9007199254740992)*((348437586779514700475067630180842053206482623665*cos(q1L))/2993155353253689176481146537402947624255349848014848 + (127834588709863499538908289888301307693646315855*sin(q1L))/5986310706507378352962293074805895248510699696029696 - (67682029681889335677290557259385*cos(q2L)*((5148155107303929*cos(q1L))/9007199254740992 + (1888752292310023*sin(q1L))/18014398509481984))/332306998946228968225951765070086144 + (9007199067919185*sin(q2L)*((1888752292310023*cos(q1L))/18014398509481984 - (5148155107303929*sin(q1L))/9007199254740992))/9007199254740992) + (7514214926474921*cos(q4L)*((9007199067919185*cos(q3L)*((46370457884011341126541404977865*cos(q1L))/81129638414606681695789005144064 + (17012367886825063216155529491255*sin(q1L))/162259276829213363391578010288128))/9007199254740992 + (7514214926474921*cos(q3L)*((7514214926474921*cos(q2L)*((5148155107303929*cos(q1L))/9007199254740992 + (1888752292310023*sin(q1L))/18014398509481984))/36893488147419103232 - sin(q2L)*((1888752292310023*cos(q1L))/18014398509481984 - (5148155107303929*sin(q1L))/9007199254740992)))/36893488147419103232 + sin(q3L)*(cos(q2L)*((1888752292310023*cos(q1L))/18014398509481984 - (5148155107303929*sin(q1L))/9007199254740992) + (7514214926474921*sin(q2L)*((5148155107303929*cos(q1L))/9007199254740992 + (1888752292310023*sin(q1L))/18014398509481984))/36893488147419103232)))/36893488147419103232))/36893488147419103232000 + (27*cos(q5L)*(((7514214926474921*cos(q4L))/36893488147419103232 + (4503599440548691*sin(q4L))/4503599627370496)*((9007199067919185*sin(q3L)*((46370457884011341126541404977865*cos(q1L))/81129638414606681695789005144064 + (17012367886825063216155529491255*sin(q1L))/162259276829213363391578010288128))/9007199254740992 - cos(q3L)*(cos(q2L)*((1888752292310023*cos(q1L))/18014398509481984 - (5148155107303929*sin(q1L))/9007199254740992) + (7514214926474921*sin(q2L)*((5148155107303929*cos(q1L))/9007199254740992 + (1888752292310023*sin(q1L))/18014398509481984))/36893488147419103232) + (7514214926474921*sin(q3L)*((7514214926474921*cos(q2L)*((5148155107303929*cos(q1L))/9007199254740992 + (1888752292310023*sin(q1L))/18014398509481984))/36893488147419103232 - sin(q2L)*((1888752292310023*cos(q1L))/18014398509481984 - (5148155107303929*sin(q1L))/9007199254740992)))/36893488147419103232) - ((9007199067919185*cos(q4L))/9007199254740992 - (234819211581865*sin(q4L))/1152921504606846976)*((348437586779514700475067630180842053206482623665*cos(q1L))/2993155353253689176481146537402947624255349848014848 + (127834588709863499538908289888301307693646315855*sin(q1L))/5986310706507378352962293074805895248510699696029696 - (67682029681889335677290557259385*cos(q2L)*((5148155107303929*cos(q1L))/9007199254740992 + (1888752292310023*sin(q1L))/18014398509481984))/332306998946228968225951765070086144 + (9007199067919185*sin(q2L)*((1888752292310023*cos(q1L))/18014398509481984 - (5148155107303929*sin(q1L))/9007199254740992))/9007199254740992) + (7514214926474921*sin(q4L)*((9007199067919185*cos(q3L)*((46370457884011341126541404977865*cos(q1L))/81129638414606681695789005144064 + (17012367886825063216155529491255*sin(q1L))/162259276829213363391578010288128))/9007199254740992 + (7514214926474921*cos(q3L)*((7514214926474921*cos(q2L)*((5148155107303929*cos(q1L))/9007199254740992 + (1888752292310023*sin(q1L))/18014398509481984))/36893488147419103232 - sin(q2L)*((1888752292310023*cos(q1L))/18014398509481984 - (5148155107303929*sin(q1L))/9007199254740992)))/36893488147419103232 + sin(q3L)*(cos(q2L)*((1888752292310023*cos(q1L))/18014398509481984 - (5148155107303929*sin(q1L))/9007199254740992) + (7514214926474921*sin(q2L)*((5148155107303929*cos(q1L))/9007199254740992 + (1888752292310023*sin(q1L))/18014398509481984))/36893488147419103232)))/36893488147419103232))/1000 + (94754841554645069948206780163139*sin(q5L)*(((7514214926474921*cos(q4L))/36893488147419103232 + (4503599440548691*sin(q4L))/4503599627370496)*((9007199067919185*sin(q3L)*((46370457884011341126541404977865*cos(q1L))/81129638414606681695789005144064 + (17012367886825063216155529491255*sin(q1L))/162259276829213363391578010288128))/9007199254740992 - cos(q3L)*(cos(q2L)*((1888752292310023*cos(q1L))/18014398509481984 - (5148155107303929*sin(q1L))/9007199254740992) + (7514214926474921*sin(q2L)*((5148155107303929*cos(q1L))/9007199254740992 + (1888752292310023*sin(q1L))/18014398509481984))/36893488147419103232) + (7514214926474921*sin(q3L)*((7514214926474921*cos(q2L)*((5148155107303929*cos(q1L))/9007199254740992 + (1888752292310023*sin(q1L))/18014398509481984))/36893488147419103232 - sin(q2L)*((1888752292310023*cos(q1L))/18014398509481984 - (5148155107303929*sin(q1L))/9007199254740992)))/36893488147419103232) - ((9007199067919185*cos(q4L))/9007199254740992 - (234819211581865*sin(q4L))/1152921504606846976)*((348437586779514700475067630180842053206482623665*cos(q1L))/2993155353253689176481146537402947624255349848014848 + (127834588709863499538908289888301307693646315855*sin(q1L))/5986310706507378352962293074805895248510699696029696 - (67682029681889335677290557259385*cos(q2L)*((5148155107303929*cos(q1L))/9007199254740992 + (1888752292310023*sin(q1L))/18014398509481984))/332306998946228968225951765070086144 + (9007199067919185*sin(q2L)*((1888752292310023*cos(q1L))/18014398509481984 - (5148155107303929*sin(q1L))/9007199254740992))/9007199254740992) + (7514214926474921*sin(q4L)*((9007199067919185*cos(q3L)*((46370457884011341126541404977865*cos(q1L))/81129638414606681695789005144064 + (17012367886825063216155529491255*sin(q1L))/162259276829213363391578010288128))/9007199254740992 + (7514214926474921*cos(q3L)*((7514214926474921*cos(q2L)*((5148155107303929*cos(q1L))/9007199254740992 + (1888752292310023*sin(q1L))/18014398509481984))/36893488147419103232 - sin(q2L)*((1888752292310023*cos(q1L))/18014398509481984 - (5148155107303929*sin(q1L))/9007199254740992)))/36893488147419103232 + sin(q3L)*(cos(q2L)*((1888752292310023*cos(q1L))/18014398509481984 - (5148155107303929*sin(q1L))/9007199254740992) + (7514214926474921*sin(q2L)*((5148155107303929*cos(q1L))/9007199254740992 + (1888752292310023*sin(q1L))/18014398509481984))/36893488147419103232)))/36893488147419103232))/66461399789245793645190353014017228800 - (610321541873521657855151997354401418608858870661075444886782706002880706727*cos(q4L)*((9007199067919185*cos(q3L)*((46370457884011341126541404977865*cos(q1L))/81129638414606681695789005144064 + (17012367886825063216155529491255*sin(q1L))/162259276829213363391578010288128))/9007199254740992 + (7514214926474921*cos(q3L)*((7514214926474921*cos(q2L)*((5148155107303929*cos(q1L))/9007199254740992 + (1888752292310023*sin(q1L))/18014398509481984))/36893488147419103232 - sin(q2L)*((1888752292310023*cos(q1L))/18014398509481984 - (5148155107303929*sin(q1L))/9007199254740992)))/36893488147419103232 + sin(q3L)*(cos(q2L)*((1888752292310023*cos(q1L))/18014398509481984 - (5148155107303929*sin(q1L))/9007199254740992) + (7514214926474921*sin(q2L)*((5148155107303929*cos(q1L))/9007199254740992 + (1888752292310023*sin(q1L))/18014398509481984))/36893488147419103232)))/11307821214581659709333104004754678501295896940003961331978279688272766566400000 - (807520961047489018778067709720399904923771262077295170375712179706208528987338271217011451790113918662491539890779991*cos(q2L)*((5148155107303929*cos(q1L))/9007199254740992 + (1888752292310023*sin(q1L))/18014398509481984))/15760802478557791684911616040057445522031895708186178667179317361698288708598884244565706501953966256322651196122726400000 + (3*cos(q2L)*((1888752292310023*cos(q1L))/18014398509481984 - (5148155107303929*sin(q1L))/9007199254740992))/100 - (608651409044468601*sin(q4L)*((9007199067919185*cos(q3L)*((46370457884011341126541404977865*cos(q1L))/81129638414606681695789005144064 + (17012367886825063216155529491255*sin(q1L))/162259276829213363391578010288128))/9007199254740992 + (7514214926474921*cos(q3L)*((7514214926474921*cos(q2L)*((5148155107303929*cos(q1L))/9007199254740992 + (1888752292310023*sin(q1L))/18014398509481984))/36893488147419103232 - sin(q2L)*((1888752292310023*cos(q1L))/18014398509481984 - (5148155107303929*sin(q1L))/9007199254740992)))/36893488147419103232 + sin(q3L)*(cos(q2L)*((1888752292310023*cos(q1L))/18014398509481984 - (5148155107303929*sin(q1L))/9007199254740992) + (7514214926474921*sin(q2L)*((5148155107303929*cos(q1L))/9007199254740992 + (1888752292310023*sin(q1L))/18014398509481984))/36893488147419103232)))/73786976294838206464000 + (22542644779424763*sin(q2L)*((5148155107303929*cos(q1L))/9007199254740992 + (1888752292310023*sin(q1L))/18014398509481984))/3689348814741910323200 + (107465779053290185796889472867275736954369330186921663479979246519176992895505610212310958309481948671*sin(q2L)*((1888752292310023*cos(q1L))/18014398509481984 - (5148155107303929*sin(q1L))/9007199254740992))/427197407184182016479004341233910422920540904471330553989408321564443945156128110004592417387315200000 - (584133382113593486367040631332731*cos(q6L)*((4103232012549050127002853406486981568002484640001584768985731379819526340981375*cos(q1L))/4171849679533027504677776769862406473833407270227837441302815640277772901915313574263597826048 + (1505391486473788436097625250507314324708888899597829175746983442666913297354625*sin(q1L))/8343699359066055009355553539724812947666814540455674882605631280555545803830627148527195652096 + (9007199067919185*((4503599440548691*cos(q4L))/4503599627370496 - (7514214926474921*sin(q4L))/36893488147419103232)*((9007199067919185*sin(q3L)*((46370457884011341126541404977865*cos(q1L))/81129638414606681695789005144064 + (17012367886825063216155529491255*sin(q1L))/162259276829213363391578010288128))/9007199254740992 - cos(q3L)*(cos(q2L)*((1888752292310023*cos(q1L))/18014398509481984 - (5148155107303929*sin(q1L))/9007199254740992) + (7514214926474921*sin(q2L)*((5148155107303929*cos(q1L))/9007199254740992 + (1888752292310023*sin(q1L))/18014398509481984))/36893488147419103232) + (7514214926474921*sin(q3L)*((7514214926474921*cos(q2L)*((5148155107303929*cos(q1L))/9007199254740992 + (1888752292310023*sin(q1L))/18014398509481984))/36893488147419103232 - sin(q2L)*((1888752292310023*cos(q1L))/18014398509481984 - (5148155107303929*sin(q1L))/9007199254740992)))/36893488147419103232))/9007199254740992 - (609625514665592237562888769449172969868262801225*cos(q3L)*((46370457884011341126541404977865*cos(q1L))/81129638414606681695789005144064 + (17012367886825063216155529491255*sin(q1L))/162259276829213363391578010288128))/2993155353253689176481146537402947624255349848014848 + (15893040848161638993908057577265778144967053025*sin(q3L)*((46370457884011341126541404977865*cos(q1L))/81129638414606681695789005144064 + (17012367886825063216155529491255*sin(q1L))/162259276829213363391578010288128))/383123885216472214589586756787577295904684780545900544 + (9007199067919185*((234819211581865*cos(q4L))/1152921504606846976 + (9007199067919185*sin(q4L))/9007199254740992)*((348437586779514700475067630180842053206482623665*cos(q1L))/2993155353253689176481146537402947624255349848014848 + (127834588709863499538908289888301307693646315855*sin(q1L))/5986310706507378352962293074805895248510699696029696 - (67682029681889335677290557259385*cos(q2L)*((5148155107303929*cos(q1L))/9007199254740992 + (1888752292310023*sin(q1L))/18014398509481984))/332306998946228968225951765070086144 + (9007199067919185*sin(q2L)*((1888752292310023*cos(q1L))/18014398509481984 - (5148155107303929*sin(q1L))/9007199254740992))/9007199254740992))/9007199254740992 - (1764482024691522628700660907665*cos(q3L)*(cos(q2L)*((1888752292310023*cos(q1L))/18014398509481984 - (5148155107303929*sin(q1L))/9007199254740992) + (7514214926474921*sin(q2L)*((5148155107303929*cos(q1L))/9007199254740992 + (1888752292310023*sin(q1L))/18014398509481984))/36893488147419103232))/42535295865117307932921825928971026432 - (508577317689771495245073589786522929324694383585*cos(q3L)*((7514214926474921*cos(q2L)*((5148155107303929*cos(q1L))/9007199254740992 + (1888752292310023*sin(q1L))/18014398509481984))/36893488147419103232 - sin(q2L)*((1888752292310023*cos(q1L))/18014398509481984 - (5148155107303929*sin(q1L))/9007199254740992)))/12259964326927110866866776217202473468949912977468817408 - (67682029681889335677290557259385*sin(q3L)*(cos(q2L)*((1888752292310023*cos(q1L))/18014398509481984 - (5148155107303929*sin(q1L))/9007199254740992) + (7514214926474921*sin(q2L)*((5148155107303929*cos(q1L))/9007199254740992 + (1888752292310023*sin(q1L))/18014398509481984))/36893488147419103232))/332306998946228968225951765070086144 + (13258697167433729449897784796786197386719169465*sin(q3L)*((7514214926474921*cos(q2L)*((5148155107303929*cos(q1L))/9007199254740992 + (1888752292310023*sin(q1L))/18014398509481984))/36893488147419103232 - sin(q2L)*((1888752292310023*cos(q1L))/18014398509481984 - (5148155107303929*sin(q1L))/9007199254740992)))/1569275433846670190958947355801916604025588861116008628224 + (67682029681889335677290557259385*cos(q4L)*((9007199067919185*cos(q3L)*((46370457884011341126541404977865*cos(q1L))/81129638414606681695789005144064 + (17012367886825063216155529491255*sin(q1L))/162259276829213363391578010288128))/9007199254740992 + (7514214926474921*cos(q3L)*((7514214926474921*cos(q2L)*((5148155107303929*cos(q1L))/9007199254740992 + (1888752292310023*sin(q1L))/18014398509481984))/36893488147419103232 - sin(q2L)*((1888752292310023*cos(q1L))/18014398509481984 - (5148155107303929*sin(q1L))/9007199254740992)))/36893488147419103232 + sin(q3L)*(cos(q2L)*((1888752292310023*cos(q1L))/18014398509481984 - (5148155107303929*sin(q1L))/9007199254740992) + (7514214926474921*sin(q2L)*((5148155107303929*cos(q1L))/9007199254740992 + (1888752292310023*sin(q1L))/18014398509481984))/36893488147419103232)))/332306998946228968225951765070086144 - (797029601289130257223357069404502671534492977261568326111352375*cos(q2L)*((5148155107303929*cos(q1L))/9007199254740992 + (1888752292310023*sin(q1L))/18014398509481984))/463168356949264781694283940034751631413079938662562256157830336031652518559744 + (106069577339469832923929692356850887620017617375*sin(q2L)*((1888752292310023*cos(q1L))/18014398509481984 - (5148155107303929*sin(q1L))/9007199254740992))/12554203470773361527671578846415332832204710888928069025792))/16225927682921336339157801028812800 - (170695144106365826517608855445768431563113584343*cos(q5L)*((546062636309760713610973115066597791006802105742542518556166375*cos(q1L))/113078212145816597093331040047546785012958969400039613319782796882727665664 + (200339157344278917575443724098432450908090682630030995291449625*sin(q1L))/226156424291633194186662080095093570025917938800079226639565593765455331328 - (81129635049124235038645691064225*cos(q3L)*((46370457884011341126541404977865*cos(q1L))/81129638414606681695789005144064 + (17012367886825063216155529491255*sin(q1L))/162259276829213363391578010288128))/81129638414606681695789005144064 + (2115063383689692319117831580025*sin(q3L)*((46370457884011341126541404977865*cos(q1L))/81129638414606681695789005144064 + (17012367886825063216155529491255*sin(q1L))/162259276829213363391578010288128))/10384593717069655257060992658440192 - (234819211581865*cos(q3L)*(cos(q2L)*((1888752292310023*cos(q1L))/18014398509481984 - (5148155107303929*sin(q1L))/9007199254740992) + (7514214926474921*sin(q2L)*((5148155107303929*cos(q1L))/9007199254740992 + (1888752292310023*sin(q1L))/18014398509481984))/36893488147419103232))/1152921504606846976 - (67682029681889335677290557259385*cos(q3L)*((7514214926474921*cos(q2L)*((5148155107303929*cos(q1L))/9007199254740992 + (1888752292310023*sin(q1L))/18014398509481984))/36893488147419103232 - sin(q2L)*((1888752292310023*cos(q1L))/18014398509481984 - (5148155107303929*sin(q1L))/9007199254740992)))/332306998946228968225951765070086144 - (9007199067919185*sin(q3L)*(cos(q2L)*((1888752292310023*cos(q1L))/18014398509481984 - (5148155107303929*sin(q1L))/9007199254740992) + (7514214926474921*sin(q2L)*((5148155107303929*cos(q1L))/9007199254740992 + (1888752292310023*sin(q1L))/18014398509481984))/36893488147419103232))/9007199254740992 + (1764482024691522628700660907665*sin(q3L)*((7514214926474921*cos(q2L)*((5148155107303929*cos(q1L))/9007199254740992 + (1888752292310023*sin(q1L))/18014398509481984))/36893488147419103232 - sin(q2L)*((1888752292310023*cos(q1L))/18014398509481984 - (5148155107303929*sin(q1L))/9007199254740992)))/42535295865117307932921825928971026432 - (106069577339469832923929692356850887620017617375*cos(q2L)*((5148155107303929*cos(q1L))/9007199254740992 + (1888752292310023*sin(q1L))/18014398509481984))/12554203470773361527671578846415332832204710888928069025792 + (14115856197532180673579726082375*sin(q2L)*((1888752292310023*cos(q1L))/18014398509481984 - (5148155107303929*sin(q1L))/9007199254740992))/340282366920938463463374607431768211456))/119726214130147567059245861496117904970213993920593920 - (48638874966763599*sin(q6L)*((4103232012549050127002853406486981568002484640001584768985731379819526340981375*cos(q1L))/4171849679533027504677776769862406473833407270227837441302815640277772901915313574263597826048 + (1505391486473788436097625250507314324708888899597829175746983442666913297354625*sin(q1L))/8343699359066055009355553539724812947666814540455674882605631280555545803830627148527195652096 + (9007199067919185*((4503599440548691*cos(q4L))/4503599627370496 - (7514214926474921*sin(q4L))/36893488147419103232)*((9007199067919185*sin(q3L)*((46370457884011341126541404977865*cos(q1L))/81129638414606681695789005144064 + (17012367886825063216155529491255*sin(q1L))/162259276829213363391578010288128))/9007199254740992 - cos(q3L)*(cos(q2L)*((1888752292310023*cos(q1L))/18014398509481984 - (5148155107303929*sin(q1L))/9007199254740992) + (7514214926474921*sin(q2L)*((5148155107303929*cos(q1L))/9007199254740992 + (1888752292310023*sin(q1L))/18014398509481984))/36893488147419103232) + (7514214926474921*sin(q3L)*((7514214926474921*cos(q2L)*((5148155107303929*cos(q1L))/9007199254740992 + (1888752292310023*sin(q1L))/18014398509481984))/36893488147419103232 - sin(q2L)*((1888752292310023*cos(q1L))/18014398509481984 - (5148155107303929*sin(q1L))/9007199254740992)))/36893488147419103232))/9007199254740992 - (609625514665592237562888769449172969868262801225*cos(q3L)*((46370457884011341126541404977865*cos(q1L))/81129638414606681695789005144064 + (17012367886825063216155529491255*sin(q1L))/162259276829213363391578010288128))/2993155353253689176481146537402947624255349848014848 + (15893040848161638993908057577265778144967053025*sin(q3L)*((46370457884011341126541404977865*cos(q1L))/81129638414606681695789005144064 + (17012367886825063216155529491255*sin(q1L))/162259276829213363391578010288128))/383123885216472214589586756787577295904684780545900544 + (9007199067919185*((234819211581865*cos(q4L))/1152921504606846976 + (9007199067919185*sin(q4L))/9007199254740992)*((348437586779514700475067630180842053206482623665*cos(q1L))/2993155353253689176481146537402947624255349848014848 + (127834588709863499538908289888301307693646315855*sin(q1L))/5986310706507378352962293074805895248510699696029696 - (67682029681889335677290557259385*cos(q2L)*((5148155107303929*cos(q1L))/9007199254740992 + (1888752292310023*sin(q1L))/18014398509481984))/332306998946228968225951765070086144 + (9007199067919185*sin(q2L)*((1888752292310023*cos(q1L))/18014398509481984 - (5148155107303929*sin(q1L))/9007199254740992))/9007199254740992))/9007199254740992 - (1764482024691522628700660907665*cos(q3L)*(cos(q2L)*((1888752292310023*cos(q1L))/18014398509481984 - (5148155107303929*sin(q1L))/9007199254740992) + (7514214926474921*sin(q2L)*((5148155107303929*cos(q1L))/9007199254740992 + (1888752292310023*sin(q1L))/18014398509481984))/36893488147419103232))/42535295865117307932921825928971026432 - (508577317689771495245073589786522929324694383585*cos(q3L)*((7514214926474921*cos(q2L)*((5148155107303929*cos(q1L))/9007199254740992 + (1888752292310023*sin(q1L))/18014398509481984))/36893488147419103232 - sin(q2L)*((1888752292310023*cos(q1L))/18014398509481984 - (5148155107303929*sin(q1L))/9007199254740992)))/12259964326927110866866776217202473468949912977468817408 - (67682029681889335677290557259385*sin(q3L)*(cos(q2L)*((1888752292310023*cos(q1L))/18014398509481984 - (5148155107303929*sin(q1L))/9007199254740992) + (7514214926474921*sin(q2L)*((5148155107303929*cos(q1L))/9007199254740992 + (1888752292310023*sin(q1L))/18014398509481984))/36893488147419103232))/332306998946228968225951765070086144 + (13258697167433729449897784796786197386719169465*sin(q3L)*((7514214926474921*cos(q2L)*((5148155107303929*cos(q1L))/9007199254740992 + (1888752292310023*sin(q1L))/18014398509481984))/36893488147419103232 - sin(q2L)*((1888752292310023*cos(q1L))/18014398509481984 - (5148155107303929*sin(q1L))/9007199254740992)))/1569275433846670190958947355801916604025588861116008628224 + (67682029681889335677290557259385*cos(q4L)*((9007199067919185*cos(q3L)*((46370457884011341126541404977865*cos(q1L))/81129638414606681695789005144064 + (17012367886825063216155529491255*sin(q1L))/162259276829213363391578010288128))/9007199254740992 + (7514214926474921*cos(q3L)*((7514214926474921*cos(q2L)*((5148155107303929*cos(q1L))/9007199254740992 + (1888752292310023*sin(q1L))/18014398509481984))/36893488147419103232 - sin(q2L)*((1888752292310023*cos(q1L))/18014398509481984 - (5148155107303929*sin(q1L))/9007199254740992)))/36893488147419103232 + sin(q3L)*(cos(q2L)*((1888752292310023*cos(q1L))/18014398509481984 - (5148155107303929*sin(q1L))/9007199254740992) + (7514214926474921*sin(q2L)*((5148155107303929*cos(q1L))/9007199254740992 + (1888752292310023*sin(q1L))/18014398509481984))/36893488147419103232)))/332306998946228968225951765070086144 - (797029601289130257223357069404502671534492977261568326111352375*cos(q2L)*((5148155107303929*cos(q1L))/9007199254740992 + (1888752292310023*sin(q1L))/18014398509481984))/463168356949264781694283940034751631413079938662562256157830336031652518559744 + (106069577339469832923929692356850887620017617375*sin(q2L)*((1888752292310023*cos(q1L))/18014398509481984 - (5148155107303929*sin(q1L))/9007199254740992))/12554203470773361527671578846415332832204710888928069025792))/1801439850948198400 + (48638874966763599*sin(q5L)*((546062636309760713610973115066597791006802105742542518556166375*cos(q1L))/113078212145816597093331040047546785012958969400039613319782796882727665664 + (200339157344278917575443724098432450908090682630030995291449625*sin(q1L))/226156424291633194186662080095093570025917938800079226639565593765455331328 - (81129635049124235038645691064225*cos(q3L)*((46370457884011341126541404977865*cos(q1L))/81129638414606681695789005144064 + (17012367886825063216155529491255*sin(q1L))/162259276829213363391578010288128))/81129638414606681695789005144064 + (2115063383689692319117831580025*sin(q3L)*((46370457884011341126541404977865*cos(q1L))/81129638414606681695789005144064 + (17012367886825063216155529491255*sin(q1L))/162259276829213363391578010288128))/10384593717069655257060992658440192 - (234819211581865*cos(q3L)*(cos(q2L)*((1888752292310023*cos(q1L))/18014398509481984 - (5148155107303929*sin(q1L))/9007199254740992) + (7514214926474921*sin(q2L)*((5148155107303929*cos(q1L))/9007199254740992 + (1888752292310023*sin(q1L))/18014398509481984))/36893488147419103232))/1152921504606846976 - (67682029681889335677290557259385*cos(q3L)*((7514214926474921*cos(q2L)*((5148155107303929*cos(q1L))/9007199254740992 + (1888752292310023*sin(q1L))/18014398509481984))/36893488147419103232 - sin(q2L)*((1888752292310023*cos(q1L))/18014398509481984 - (5148155107303929*sin(q1L))/9007199254740992)))/332306998946228968225951765070086144 - (9007199067919185*sin(q3L)*(cos(q2L)*((1888752292310023*cos(q1L))/18014398509481984 - (5148155107303929*sin(q1L))/9007199254740992) + (7514214926474921*sin(q2L)*((5148155107303929*cos(q1L))/9007199254740992 + (1888752292310023*sin(q1L))/18014398509481984))/36893488147419103232))/9007199254740992 + (1764482024691522628700660907665*sin(q3L)*((7514214926474921*cos(q2L)*((5148155107303929*cos(q1L))/9007199254740992 + (1888752292310023*sin(q1L))/18014398509481984))/36893488147419103232 - sin(q2L)*((1888752292310023*cos(q1L))/18014398509481984 - (5148155107303929*sin(q1L))/9007199254740992)))/42535295865117307932921825928971026432 - (106069577339469832923929692356850887620017617375*cos(q2L)*((5148155107303929*cos(q1L))/9007199254740992 + (1888752292310023*sin(q1L))/18014398509481984))/12554203470773361527671578846415332832204710888928069025792 + (14115856197532180673579726082375*sin(q2L)*((1888752292310023*cos(q1L))/18014398509481984 - (5148155107303929*sin(q1L))/9007199254740992))/340282366920938463463374607431768211456))/1801439850948198400, (48638874966763599*sin(q5L)*((14115856197532180673579726082375*cos(q2L)*((5148155107303929*cos(q1L))/9007199254740992 + (1888752292310023*sin(q1L))/18014398509481984))/340282366920938463463374607431768211456 - (233003667623740560033643537092505706768317191960312467162596875*sin(q2L))/6901746346790563787434755862277025452451108972170386555162524223799296 + (234819211581865*cos(q3L)*((16506520352940097956833727997725*cos(q2L))/20282409603651670423947251286016 + (7514214926474921*cos(q2L)*((1888752292310023*cos(q1L))/18014398509481984 - (5148155107303929*sin(q1L))/9007199254740992))/36893488147419103232 + sin(q2L)*((5148155107303929*cos(q1L))/9007199254740992 + (1888752292310023*sin(q1L))/18014398509481984)))/1152921504606846976 - (106069577339469832923929692356850887620017617375*sin(q2L)*((1888752292310023*cos(q1L))/18014398509481984 - (5148155107303929*sin(q1L))/9007199254740992))/12554203470773361527671578846415332832204710888928069025792 + (9007199067919185*sin(q3L)*((16506520352940097956833727997725*cos(q2L))/20282409603651670423947251286016 + (7514214926474921*cos(q2L)*((1888752292310023*cos(q1L))/18014398509481984 - (5148155107303929*sin(q1L))/9007199254740992))/36893488147419103232 + sin(q2L)*((5148155107303929*cos(q1L))/9007199254740992 + (1888752292310023*sin(q1L))/18014398509481984)))/9007199254740992 - (67682029681889335677290557259385*cos(q3L)*((16506520352940097956833727997725*sin(q2L))/20282409603651670423947251286016 - cos(q2L)*((5148155107303929*cos(q1L))/9007199254740992 + (1888752292310023*sin(q1L))/18014398509481984) + (7514214926474921*sin(q2L)*((1888752292310023*cos(q1L))/18014398509481984 - (5148155107303929*sin(q1L))/9007199254740992))/36893488147419103232))/332306998946228968225951765070086144 + (1764482024691522628700660907665*sin(q3L)*((16506520352940097956833727997725*sin(q2L))/20282409603651670423947251286016 - cos(q2L)*((5148155107303929*cos(q1L))/9007199254740992 + (1888752292310023*sin(q1L))/18014398509481984) + (7514214926474921*sin(q2L)*((1888752292310023*cos(q1L))/18014398509481984 - (5148155107303929*sin(q1L))/9007199254740992))/36893488147419103232))/42535295865117307932921825928971026432))/1801439850948198400 - (70955442767507924149430414788592465764454924696039647595449074492918405062780420917918753205474800032457614998917774096940162190939*sin(q2L))/346583711765101857447301773017885462929554634421977071896309947576827663475703202879996800763017447262173901370175446478621769728000 - (81222263116692158804177042061221826384594597321566869716687*((4503599440548691*cos(q4L))/4503599627370496 - (7514214926474921*sin(q4L))/36893488147419103232)*(cos(q3L)*((16506520352940097956833727997725*cos(q2L))/20282409603651670423947251286016 + (7514214926474921*cos(q2L)*((1888752292310023*cos(q1L))/18014398509481984 - (5148155107303929*sin(q1L))/9007199254740992))/36893488147419103232 + sin(q2L)*((5148155107303929*cos(q1L))/9007199254740992 + (1888752292310023*sin(q1L))/18014398509481984)) + (7514214926474921*sin(q3L)*((16506520352940097956833727997725*sin(q2L))/20282409603651670423947251286016 - cos(q2L)*((5148155107303929*cos(q1L))/9007199254740992 + (1888752292310023*sin(q1L))/18014398509481984) + (7514214926474921*sin(q2L)*((1888752292310023*cos(q1L))/18014398509481984 - (5148155107303929*sin(q1L))/9007199254740992))/36893488147419103232))/36893488147419103232))/306499108173177771671669405430061836723747824436720435200000 - (81*((7514214926474921*cos(q4L))/36893488147419103232 + (4503599440548691*sin(q4L))/4503599627370496)*(cos(q3L)*((16506520352940097956833727997725*cos(q2L))/20282409603651670423947251286016 + (7514214926474921*cos(q2L)*((1888752292310023*cos(q1L))/18014398509481984 - (5148155107303929*sin(q1L))/9007199254740992))/36893488147419103232 + sin(q2L)*((5148155107303929*cos(q1L))/9007199254740992 + (1888752292310023*sin(q1L))/18014398509481984)) + (7514214926474921*sin(q3L)*((16506520352940097956833727997725*sin(q2L))/20282409603651670423947251286016 - cos(q2L)*((5148155107303929*cos(q1L))/9007199254740992 + (1888752292310023*sin(q1L))/18014398509481984) + (7514214926474921*sin(q2L)*((1888752292310023*cos(q1L))/18014398509481984 - (5148155107303929*sin(q1L))/9007199254740992))/36893488147419103232))/36893488147419103232))/2000 - (170695144106365826517608855445768431563113584343*cos(q5L)*((14115856197532180673579726082375*cos(q2L)*((5148155107303929*cos(q1L))/9007199254740992 + (1888752292310023*sin(q1L))/18014398509481984))/340282366920938463463374607431768211456 - (233003667623740560033643537092505706768317191960312467162596875*sin(q2L))/6901746346790563787434755862277025452451108972170386555162524223799296 + (234819211581865*cos(q3L)*((16506520352940097956833727997725*cos(q2L))/20282409603651670423947251286016 + (7514214926474921*cos(q2L)*((1888752292310023*cos(q1L))/18014398509481984 - (5148155107303929*sin(q1L))/9007199254740992))/36893488147419103232 + sin(q2L)*((5148155107303929*cos(q1L))/9007199254740992 + (1888752292310023*sin(q1L))/18014398509481984)))/1152921504606846976 - (106069577339469832923929692356850887620017617375*sin(q2L)*((1888752292310023*cos(q1L))/18014398509481984 - (5148155107303929*sin(q1L))/9007199254740992))/12554203470773361527671578846415332832204710888928069025792 + (9007199067919185*sin(q3L)*((16506520352940097956833727997725*cos(q2L))/20282409603651670423947251286016 + (7514214926474921*cos(q2L)*((1888752292310023*cos(q1L))/18014398509481984 - (5148155107303929*sin(q1L))/9007199254740992))/36893488147419103232 + sin(q2L)*((5148155107303929*cos(q1L))/9007199254740992 + (1888752292310023*sin(q1L))/18014398509481984)))/9007199254740992 - (67682029681889335677290557259385*cos(q3L)*((16506520352940097956833727997725*sin(q2L))/20282409603651670423947251286016 - cos(q2L)*((5148155107303929*cos(q1L))/9007199254740992 + (1888752292310023*sin(q1L))/18014398509481984) + (7514214926474921*sin(q2L)*((1888752292310023*cos(q1L))/18014398509481984 - (5148155107303929*sin(q1L))/9007199254740992))/36893488147419103232))/332306998946228968225951765070086144 + (1764482024691522628700660907665*sin(q3L)*((16506520352940097956833727997725*sin(q2L))/20282409603651670423947251286016 - cos(q2L)*((5148155107303929*cos(q1L))/9007199254740992 + (1888752292310023*sin(q1L))/18014398509481984) + (7514214926474921*sin(q2L)*((1888752292310023*cos(q1L))/18014398509481984 - (5148155107303929*sin(q1L))/9007199254740992))/36893488147419103232))/42535295865117307932921825928971026432))/119726214130147567059245861496117904970213993920593920 - (1980782442352811754820047359727*cos(q2L))/81129638414606681695789005144064 - (81*((9007199067919185*cos(q4L))/9007199254740992 - (234819211581865*sin(q4L))/1152921504606846976)*((148677514737591106934298605035692608392163854125*sin(q2L))/182687704666362864775460604089535377456991567872 - (9007199067919185*cos(q2L)*((5148155107303929*cos(q1L))/9007199254740992 + (1888752292310023*sin(q1L))/18014398509481984))/9007199254740992 + (67682029681889335677290557259385*sin(q2L)*((1888752292310023*cos(q1L))/18014398509481984 - (5148155107303929*sin(q1L))/9007199254740992))/332306998946228968225951765070086144))/2000 + (81222263116692158804177042061221826384594597321566869716687*((234819211581865*cos(q4L))/1152921504606846976 + (9007199067919185*sin(q4L))/9007199254740992)*((148677514737591106934298605035692608392163854125*sin(q2L))/182687704666362864775460604089535377456991567872 - (9007199067919185*cos(q2L)*((5148155107303929*cos(q1L))/9007199254740992 + (1888752292310023*sin(q1L))/18014398509481984))/9007199254740992 + (67682029681889335677290557259385*sin(q2L)*((1888752292310023*cos(q1L))/18014398509481984 - (5148155107303929*sin(q1L))/9007199254740992))/332306998946228968225951765070086144))/306499108173177771671669405430061836723747824436720435200000 - (712008244765680093343103025701132101054572137019*cos(q5L)*(((234819211581865*cos(q4L))/1152921504606846976 + (9007199067919185*sin(q4L))/9007199254740992)*((148677514737591106934298605035692608392163854125*sin(q2L))/182687704666362864775460604089535377456991567872 - (9007199067919185*cos(q2L)*((5148155107303929*cos(q1L))/9007199254740992 + (1888752292310023*sin(q1L))/18014398509481984))/9007199254740992 + (67682029681889335677290557259385*sin(q2L)*((1888752292310023*cos(q1L))/18014398509481984 - (5148155107303929*sin(q1L))/9007199254740992))/332306998946228968225951765070086144) - ((4503599440548691*cos(q4L))/4503599627370496 - (7514214926474921*sin(q4L))/36893488147419103232)*(cos(q3L)*((16506520352940097956833727997725*cos(q2L))/20282409603651670423947251286016 + (7514214926474921*cos(q2L)*((1888752292310023*cos(q1L))/18014398509481984 - (5148155107303929*sin(q1L))/9007199254740992))/36893488147419103232 + sin(q2L)*((5148155107303929*cos(q1L))/9007199254740992 + (1888752292310023*sin(q1L))/18014398509481984)) + (7514214926474921*sin(q3L)*((16506520352940097956833727997725*sin(q2L))/20282409603651670423947251286016 - cos(q2L)*((5148155107303929*cos(q1L))/9007199254740992 + (1888752292310023*sin(q1L))/18014398509481984) + (7514214926474921*sin(q2L)*((1888752292310023*cos(q1L))/18014398509481984 - (5148155107303929*sin(q1L))/9007199254740992))/36893488147419103232))/36893488147419103232) + (7514214926474921*cos(q4L)*(sin(q3L)*((16506520352940097956833727997725*cos(q2L))/20282409603651670423947251286016 + (7514214926474921*cos(q2L)*((1888752292310023*cos(q1L))/18014398509481984 - (5148155107303929*sin(q1L))/9007199254740992))/36893488147419103232 + sin(q2L)*((5148155107303929*cos(q1L))/9007199254740992 + (1888752292310023*sin(q1L))/18014398509481984)) - (7514214926474921*cos(q3L)*((16506520352940097956833727997725*sin(q2L))/20282409603651670423947251286016 - cos(q2L)*((5148155107303929*cos(q1L))/9007199254740992 + (1888752292310023*sin(q1L))/18014398509481984) + (7514214926474921*sin(q2L)*((1888752292310023*cos(q1L))/18014398509481984 - (5148155107303929*sin(q1L))/9007199254740992))/36893488147419103232))/36893488147419103232))/36893488147419103232))/2451992865385422173373355243440494693789982595493763481600 + (584133382113593486367040631332731*cos(q6L)*((1750839637181712602987937819095679046818178170494703109500053864263283920471875*sin(q2L))/254629497041810760783555711051172270131433549208242031329517556169297662470417088272924672 - (9007199067919185*((4503599440548691*cos(q4L))/4503599627370496 - (7514214926474921*sin(q4L))/36893488147419103232)*(cos(q3L)*((16506520352940097956833727997725*cos(q2L))/20282409603651670423947251286016 + (7514214926474921*cos(q2L)*((1888752292310023*cos(q1L))/18014398509481984 - (5148155107303929*sin(q1L))/9007199254740992))/36893488147419103232 + sin(q2L)*((5148155107303929*cos(q1L))/9007199254740992 + (1888752292310023*sin(q1L))/18014398509481984)) + (7514214926474921*sin(q3L)*((16506520352940097956833727997725*sin(q2L))/20282409603651670423947251286016 - cos(q2L)*((5148155107303929*cos(q1L))/9007199254740992 + (1888752292310023*sin(q1L))/18014398509481984) + (7514214926474921*sin(q2L)*((1888752292310023*cos(q1L))/18014398509481984 - (5148155107303929*sin(q1L))/9007199254740992))/36893488147419103232))/36893488147419103232))/9007199254740992 + (9007199067919185*((234819211581865*cos(q4L))/1152921504606846976 + (9007199067919185*sin(q4L))/9007199254740992)*((148677514737591106934298605035692608392163854125*sin(q2L))/182687704666362864775460604089535377456991567872 - (9007199067919185*cos(q2L)*((5148155107303929*cos(q1L))/9007199254740992 + (1888752292310023*sin(q1L))/18014398509481984))/9007199254740992 + (67682029681889335677290557259385*sin(q2L)*((1888752292310023*cos(q1L))/18014398509481984 - (5148155107303929*sin(q1L))/9007199254740992))/332306998946228968225951765070086144))/9007199254740992 - (106069577339469832923929692356850887620017617375*cos(q2L)*((5148155107303929*cos(q1L))/9007199254740992 + (1888752292310023*sin(q1L))/18014398509481984))/12554203470773361527671578846415332832204710888928069025792 + (67682029681889335677290557259385*cos(q4L)*(sin(q3L)*((16506520352940097956833727997725*cos(q2L))/20282409603651670423947251286016 + (7514214926474921*cos(q2L)*((1888752292310023*cos(q1L))/18014398509481984 - (5148155107303929*sin(q1L))/9007199254740992))/36893488147419103232 + sin(q2L)*((5148155107303929*cos(q1L))/9007199254740992 + (1888752292310023*sin(q1L))/18014398509481984)) - (7514214926474921*cos(q3L)*((16506520352940097956833727997725*sin(q2L))/20282409603651670423947251286016 - cos(q2L)*((5148155107303929*cos(q1L))/9007199254740992 + (1888752292310023*sin(q1L))/18014398509481984) + (7514214926474921*sin(q2L)*((1888752292310023*cos(q1L))/18014398509481984 - (5148155107303929*sin(q1L))/9007199254740992))/36893488147419103232))/36893488147419103232))/332306998946228968225951765070086144 - (1764482024691522628700660907665*cos(q3L)*((16506520352940097956833727997725*cos(q2L))/20282409603651670423947251286016 + (7514214926474921*cos(q2L)*((1888752292310023*cos(q1L))/18014398509481984 - (5148155107303929*sin(q1L))/9007199254740992))/36893488147419103232 + sin(q2L)*((5148155107303929*cos(q1L))/9007199254740992 + (1888752292310023*sin(q1L))/18014398509481984)))/42535295865117307932921825928971026432 + (797029601289130257223357069404502671534492977261568326111352375*sin(q2L)*((1888752292310023*cos(q1L))/18014398509481984 - (5148155107303929*sin(q1L))/9007199254740992))/463168356949264781694283940034751631413079938662562256157830336031652518559744 - (67682029681889335677290557259385*sin(q3L)*((16506520352940097956833727997725*cos(q2L))/20282409603651670423947251286016 + (7514214926474921*cos(q2L)*((1888752292310023*cos(q1L))/18014398509481984 - (5148155107303929*sin(q1L))/9007199254740992))/36893488147419103232 + sin(q2L)*((5148155107303929*cos(q1L))/9007199254740992 + (1888752292310023*sin(q1L))/18014398509481984)))/332306998946228968225951765070086144 + (508577317689771495245073589786522929324694383585*cos(q3L)*((16506520352940097956833727997725*sin(q2L))/20282409603651670423947251286016 - cos(q2L)*((5148155107303929*cos(q1L))/9007199254740992 + (1888752292310023*sin(q1L))/18014398509481984) + (7514214926474921*sin(q2L)*((1888752292310023*cos(q1L))/18014398509481984 - (5148155107303929*sin(q1L))/9007199254740992))/36893488147419103232))/12259964326927110866866776217202473468949912977468817408 - (13258697167433729449897784796786197386719169465*sin(q3L)*((16506520352940097956833727997725*sin(q2L))/20282409603651670423947251286016 - cos(q2L)*((5148155107303929*cos(q1L))/9007199254740992 + (1888752292310023*sin(q1L))/18014398509481984) + (7514214926474921*sin(q2L)*((1888752292310023*cos(q1L))/18014398509481984 - (5148155107303929*sin(q1L))/9007199254740992))/36893488147419103232))/1569275433846670190958947355801916604025588861116008628224))/16225927682921336339157801028812800 + (107465779053290185796889472867275736954369330186921663479979246519176992895505610212310958309481948671*cos(q2L)*((5148155107303929*cos(q1L))/9007199254740992 + (1888752292310023*sin(q1L))/18014398509481984))/427197407184182016479004341233910422920540904471330553989408321564443945156128110004592417387315200000 - (22542644779424763*cos(q2L)*((1888752292310023*cos(q1L))/18014398509481984 - (5148155107303929*sin(q1L))/9007199254740992))/3689348814741910323200 + (610321541873521657855151997354401418608858870661075444886782706002880706727*cos(q4L)*(sin(q3L)*((16506520352940097956833727997725*cos(q2L))/20282409603651670423947251286016 + (7514214926474921*cos(q2L)*((1888752292310023*cos(q1L))/18014398509481984 - (5148155107303929*sin(q1L))/9007199254740992))/36893488147419103232 + sin(q2L)*((5148155107303929*cos(q1L))/9007199254740992 + (1888752292310023*sin(q1L))/18014398509481984)) - (7514214926474921*cos(q3L)*((16506520352940097956833727997725*sin(q2L))/20282409603651670423947251286016 - cos(q2L)*((5148155107303929*cos(q1L))/9007199254740992 + (1888752292310023*sin(q1L))/18014398509481984) + (7514214926474921*sin(q2L)*((1888752292310023*cos(q1L))/18014398509481984 - (5148155107303929*sin(q1L))/9007199254740992))/36893488147419103232))/36893488147419103232))/11307821214581659709333104004754678501295896940003961331978279688272766566400000 + (27*cos(q5L)*(((7514214926474921*cos(q4L))/36893488147419103232 + (4503599440548691*sin(q4L))/4503599627370496)*(cos(q3L)*((16506520352940097956833727997725*cos(q2L))/20282409603651670423947251286016 + (7514214926474921*cos(q2L)*((1888752292310023*cos(q1L))/18014398509481984 - (5148155107303929*sin(q1L))/9007199254740992))/36893488147419103232 + sin(q2L)*((5148155107303929*cos(q1L))/9007199254740992 + (1888752292310023*sin(q1L))/18014398509481984)) + (7514214926474921*sin(q3L)*((16506520352940097956833727997725*sin(q2L))/20282409603651670423947251286016 - cos(q2L)*((5148155107303929*cos(q1L))/9007199254740992 + (1888752292310023*sin(q1L))/18014398509481984) + (7514214926474921*sin(q2L)*((1888752292310023*cos(q1L))/18014398509481984 - (5148155107303929*sin(q1L))/9007199254740992))/36893488147419103232))/36893488147419103232) + ((9007199067919185*cos(q4L))/9007199254740992 - (234819211581865*sin(q4L))/1152921504606846976)*((148677514737591106934298605035692608392163854125*sin(q2L))/182687704666362864775460604089535377456991567872 - (9007199067919185*cos(q2L)*((5148155107303929*cos(q1L))/9007199254740992 + (1888752292310023*sin(q1L))/18014398509481984))/9007199254740992 + (67682029681889335677290557259385*sin(q2L)*((1888752292310023*cos(q1L))/18014398509481984 - (5148155107303929*sin(q1L))/9007199254740992))/332306998946228968225951765070086144) - (7514214926474921*sin(q4L)*(sin(q3L)*((16506520352940097956833727997725*cos(q2L))/20282409603651670423947251286016 + (7514214926474921*cos(q2L)*((1888752292310023*cos(q1L))/18014398509481984 - (5148155107303929*sin(q1L))/9007199254740992))/36893488147419103232 + sin(q2L)*((5148155107303929*cos(q1L))/9007199254740992 + (1888752292310023*sin(q1L))/18014398509481984)) - (7514214926474921*cos(q3L)*((16506520352940097956833727997725*sin(q2L))/20282409603651670423947251286016 - cos(q2L)*((5148155107303929*cos(q1L))/9007199254740992 + (1888752292310023*sin(q1L))/18014398509481984) + (7514214926474921*sin(q2L)*((1888752292310023*cos(q1L))/18014398509481984 - (5148155107303929*sin(q1L))/9007199254740992))/36893488147419103232))/36893488147419103232))/36893488147419103232))/1000 + (202883803014822867*sin(q5L)*(((234819211581865*cos(q4L))/1152921504606846976 + (9007199067919185*sin(q4L))/9007199254740992)*((148677514737591106934298605035692608392163854125*sin(q2L))/182687704666362864775460604089535377456991567872 - (9007199067919185*cos(q2L)*((5148155107303929*cos(q1L))/9007199254740992 + (1888752292310023*sin(q1L))/18014398509481984))/9007199254740992 + (67682029681889335677290557259385*sin(q2L)*((1888752292310023*cos(q1L))/18014398509481984 - (5148155107303929*sin(q1L))/9007199254740992))/332306998946228968225951765070086144) - ((4503599440548691*cos(q4L))/4503599627370496 - (7514214926474921*sin(q4L))/36893488147419103232)*(cos(q3L)*((16506520352940097956833727997725*cos(q2L))/20282409603651670423947251286016 + (7514214926474921*cos(q2L)*((1888752292310023*cos(q1L))/18014398509481984 - (5148155107303929*sin(q1L))/9007199254740992))/36893488147419103232 + sin(q2L)*((5148155107303929*cos(q1L))/9007199254740992 + (1888752292310023*sin(q1L))/18014398509481984)) + (7514214926474921*sin(q3L)*((16506520352940097956833727997725*sin(q2L))/20282409603651670423947251286016 - cos(q2L)*((5148155107303929*cos(q1L))/9007199254740992 + (1888752292310023*sin(q1L))/18014398509481984) + (7514214926474921*sin(q2L)*((1888752292310023*cos(q1L))/18014398509481984 - (5148155107303929*sin(q1L))/9007199254740992))/36893488147419103232))/36893488147419103232) + (7514214926474921*cos(q4L)*(sin(q3L)*((16506520352940097956833727997725*cos(q2L))/20282409603651670423947251286016 + (7514214926474921*cos(q2L)*((1888752292310023*cos(q1L))/18014398509481984 - (5148155107303929*sin(q1L))/9007199254740992))/36893488147419103232 + sin(q2L)*((5148155107303929*cos(q1L))/9007199254740992 + (1888752292310023*sin(q1L))/18014398509481984)) - (7514214926474921*cos(q3L)*((16506520352940097956833727997725*sin(q2L))/20282409603651670423947251286016 - cos(q2L)*((5148155107303929*cos(q1L))/9007199254740992 + (1888752292310023*sin(q1L))/18014398509481984) + (7514214926474921*sin(q2L)*((1888752292310023*cos(q1L))/18014398509481984 - (5148155107303929*sin(q1L))/9007199254740992))/36893488147419103232))/36893488147419103232))/36893488147419103232))/36893488147419103232000 + (2436553109258773196144549622003023*cos(q6L)*((9007199067919185*cos(q5L)*((14115856197532180673579726082375*cos(q2L)*((5148155107303929*cos(q1L))/9007199254740992 + (1888752292310023*sin(q1L))/18014398509481984))/340282366920938463463374607431768211456 - (233003667623740560033643537092505706768317191960312467162596875*sin(q2L))/6901746346790563787434755862277025452451108972170386555162524223799296 + (234819211581865*cos(q3L)*((16506520352940097956833727997725*cos(q2L))/20282409603651670423947251286016 + (7514214926474921*cos(q2L)*((1888752292310023*cos(q1L))/18014398509481984 - (5148155107303929*sin(q1L))/9007199254740992))/36893488147419103232 + sin(q2L)*((5148155107303929*cos(q1L))/9007199254740992 + (1888752292310023*sin(q1L))/18014398509481984)))/1152921504606846976 - (106069577339469832923929692356850887620017617375*sin(q2L)*((1888752292310023*cos(q1L))/18014398509481984 - (5148155107303929*sin(q1L))/9007199254740992))/12554203470773361527671578846415332832204710888928069025792 + (9007199067919185*sin(q3L)*((16506520352940097956833727997725*cos(q2L))/20282409603651670423947251286016 + (7514214926474921*cos(q2L)*((1888752292310023*cos(q1L))/18014398509481984 - (5148155107303929*sin(q1L))/9007199254740992))/36893488147419103232 + sin(q2L)*((5148155107303929*cos(q1L))/9007199254740992 + (1888752292310023*sin(q1L))/18014398509481984)))/9007199254740992 - (67682029681889335677290557259385*cos(q3L)*((16506520352940097956833727997725*sin(q2L))/20282409603651670423947251286016 - cos(q2L)*((5148155107303929*cos(q1L))/9007199254740992 + (1888752292310023*sin(q1L))/18014398509481984) + (7514214926474921*sin(q2L)*((1888752292310023*cos(q1L))/18014398509481984 - (5148155107303929*sin(q1L))/9007199254740992))/36893488147419103232))/332306998946228968225951765070086144 + (1764482024691522628700660907665*sin(q3L)*((16506520352940097956833727997725*sin(q2L))/20282409603651670423947251286016 - cos(q2L)*((5148155107303929*cos(q1L))/9007199254740992 + (1888752292310023*sin(q1L))/18014398509481984) + (7514214926474921*sin(q2L)*((1888752292310023*cos(q1L))/18014398509481984 - (5148155107303929*sin(q1L))/9007199254740992))/36893488147419103232))/42535295865117307932921825928971026432))/9007199254740992 + (7514214926474921*cos(q5L)*(((234819211581865*cos(q4L))/1152921504606846976 + (9007199067919185*sin(q4L))/9007199254740992)*((148677514737591106934298605035692608392163854125*sin(q2L))/182687704666362864775460604089535377456991567872 - (9007199067919185*cos(q2L)*((5148155107303929*cos(q1L))/9007199254740992 + (1888752292310023*sin(q1L))/18014398509481984))/9007199254740992 + (67682029681889335677290557259385*sin(q2L)*((1888752292310023*cos(q1L))/18014398509481984 - (5148155107303929*sin(q1L))/9007199254740992))/332306998946228968225951765070086144) - ((4503599440548691*cos(q4L))/4503599627370496 - (7514214926474921*sin(q4L))/36893488147419103232)*(cos(q3L)*((16506520352940097956833727997725*cos(q2L))/20282409603651670423947251286016 + (7514214926474921*cos(q2L)*((1888752292310023*cos(q1L))/18014398509481984 - (5148155107303929*sin(q1L))/9007199254740992))/36893488147419103232 + sin(q2L)*((5148155107303929*cos(q1L))/9007199254740992 + (1888752292310023*sin(q1L))/18014398509481984)) + (7514214926474921*sin(q3L)*((16506520352940097956833727997725*sin(q2L))/20282409603651670423947251286016 - cos(q2L)*((5148155107303929*cos(q1L))/9007199254740992 + (1888752292310023*sin(q1L))/18014398509481984) + (7514214926474921*sin(q2L)*((1888752292310023*cos(q1L))/18014398509481984 - (5148155107303929*sin(q1L))/9007199254740992))/36893488147419103232))/36893488147419103232) + (7514214926474921*cos(q4L)*(sin(q3L)*((16506520352940097956833727997725*cos(q2L))/20282409603651670423947251286016 + (7514214926474921*cos(q2L)*((1888752292310023*cos(q1L))/18014398509481984 - (5148155107303929*sin(q1L))/9007199254740992))/36893488147419103232 + sin(q2L)*((5148155107303929*cos(q1L))/9007199254740992 + (1888752292310023*sin(q1L))/18014398509481984)) - (7514214926474921*cos(q3L)*((16506520352940097956833727997725*sin(q2L))/20282409603651670423947251286016 - cos(q2L)*((5148155107303929*cos(q1L))/9007199254740992 + (1888752292310023*sin(q1L))/18014398509481984) + (7514214926474921*sin(q2L)*((1888752292310023*cos(q1L))/18014398509481984 - (5148155107303929*sin(q1L))/9007199254740992))/36893488147419103232))/36893488147419103232))/36893488147419103232))/36893488147419103232 - sin(q5L)*(((7514214926474921*cos(q4L))/36893488147419103232 + (4503599440548691*sin(q4L))/4503599627370496)*(cos(q3L)*((16506520352940097956833727997725*cos(q2L))/20282409603651670423947251286016 + (7514214926474921*cos(q2L)*((1888752292310023*cos(q1L))/18014398509481984 - (5148155107303929*sin(q1L))/9007199254740992))/36893488147419103232 + sin(q2L)*((5148155107303929*cos(q1L))/9007199254740992 + (1888752292310023*sin(q1L))/18014398509481984)) + (7514214926474921*sin(q3L)*((16506520352940097956833727997725*sin(q2L))/20282409603651670423947251286016 - cos(q2L)*((5148155107303929*cos(q1L))/9007199254740992 + (1888752292310023*sin(q1L))/18014398509481984) + (7514214926474921*sin(q2L)*((1888752292310023*cos(q1L))/18014398509481984 - (5148155107303929*sin(q1L))/9007199254740992))/36893488147419103232))/36893488147419103232) + ((9007199067919185*cos(q4L))/9007199254740992 - (234819211581865*sin(q4L))/1152921504606846976)*((148677514737591106934298605035692608392163854125*sin(q2L))/182687704666362864775460604089535377456991567872 - (9007199067919185*cos(q2L)*((5148155107303929*cos(q1L))/9007199254740992 + (1888752292310023*sin(q1L))/18014398509481984))/9007199254740992 + (67682029681889335677290557259385*sin(q2L)*((1888752292310023*cos(q1L))/18014398509481984 - (5148155107303929*sin(q1L))/9007199254740992))/332306998946228968225951765070086144) - (7514214926474921*sin(q4L)*(sin(q3L)*((16506520352940097956833727997725*cos(q2L))/20282409603651670423947251286016 + (7514214926474921*cos(q2L)*((1888752292310023*cos(q1L))/18014398509481984 - (5148155107303929*sin(q1L))/9007199254740992))/36893488147419103232 + sin(q2L)*((5148155107303929*cos(q1L))/9007199254740992 + (1888752292310023*sin(q1L))/18014398509481984)) - (7514214926474921*cos(q3L)*((16506520352940097956833727997725*sin(q2L))/20282409603651670423947251286016 - cos(q2L)*((5148155107303929*cos(q1L))/9007199254740992 + (1888752292310023*sin(q1L))/18014398509481984) + (7514214926474921*sin(q2L)*((1888752292310023*cos(q1L))/18014398509481984 - (5148155107303929*sin(q1L))/9007199254740992))/36893488147419103232))/36893488147419103232))/36893488147419103232)))/332306998946228968225951765070086144000 + (48638874966763599*sin(q6L)*((1750839637181712602987937819095679046818178170494703109500053864263283920471875*sin(q2L))/254629497041810760783555711051172270131433549208242031329517556169297662470417088272924672 - (9007199067919185*((4503599440548691*cos(q4L))/4503599627370496 - (7514214926474921*sin(q4L))/36893488147419103232)*(cos(q3L)*((16506520352940097956833727997725*cos(q2L))/20282409603651670423947251286016 + (7514214926474921*cos(q2L)*((1888752292310023*cos(q1L))/18014398509481984 - (5148155107303929*sin(q1L))/9007199254740992))/36893488147419103232 + sin(q2L)*((5148155107303929*cos(q1L))/9007199254740992 + (1888752292310023*sin(q1L))/18014398509481984)) + (7514214926474921*sin(q3L)*((16506520352940097956833727997725*sin(q2L))/20282409603651670423947251286016 - cos(q2L)*((5148155107303929*cos(q1L))/9007199254740992 + (1888752292310023*sin(q1L))/18014398509481984) + (7514214926474921*sin(q2L)*((1888752292310023*cos(q1L))/18014398509481984 - (5148155107303929*sin(q1L))/9007199254740992))/36893488147419103232))/36893488147419103232))/9007199254740992 + (9007199067919185*((234819211581865*cos(q4L))/1152921504606846976 + (9007199067919185*sin(q4L))/9007199254740992)*((148677514737591106934298605035692608392163854125*sin(q2L))/182687704666362864775460604089535377456991567872 - (9007199067919185*cos(q2L)*((5148155107303929*cos(q1L))/9007199254740992 + (1888752292310023*sin(q1L))/18014398509481984))/9007199254740992 + (67682029681889335677290557259385*sin(q2L)*((1888752292310023*cos(q1L))/18014398509481984 - (5148155107303929*sin(q1L))/9007199254740992))/332306998946228968225951765070086144))/9007199254740992 - (106069577339469832923929692356850887620017617375*cos(q2L)*((5148155107303929*cos(q1L))/9007199254740992 + (1888752292310023*sin(q1L))/18014398509481984))/12554203470773361527671578846415332832204710888928069025792 + (67682029681889335677290557259385*cos(q4L)*(sin(q3L)*((16506520352940097956833727997725*cos(q2L))/20282409603651670423947251286016 + (7514214926474921*cos(q2L)*((1888752292310023*cos(q1L))/18014398509481984 - (5148155107303929*sin(q1L))/9007199254740992))/36893488147419103232 + sin(q2L)*((5148155107303929*cos(q1L))/9007199254740992 + (1888752292310023*sin(q1L))/18014398509481984)) - (7514214926474921*cos(q3L)*((16506520352940097956833727997725*sin(q2L))/20282409603651670423947251286016 - cos(q2L)*((5148155107303929*cos(q1L))/9007199254740992 + (1888752292310023*sin(q1L))/18014398509481984) + (7514214926474921*sin(q2L)*((1888752292310023*cos(q1L))/18014398509481984 - (5148155107303929*sin(q1L))/9007199254740992))/36893488147419103232))/36893488147419103232))/332306998946228968225951765070086144 - (1764482024691522628700660907665*cos(q3L)*((16506520352940097956833727997725*cos(q2L))/20282409603651670423947251286016 + (7514214926474921*cos(q2L)*((1888752292310023*cos(q1L))/18014398509481984 - (5148155107303929*sin(q1L))/9007199254740992))/36893488147419103232 + sin(q2L)*((5148155107303929*cos(q1L))/9007199254740992 + (1888752292310023*sin(q1L))/18014398509481984)))/42535295865117307932921825928971026432 + (797029601289130257223357069404502671534492977261568326111352375*sin(q2L)*((1888752292310023*cos(q1L))/18014398509481984 - (5148155107303929*sin(q1L))/9007199254740992))/463168356949264781694283940034751631413079938662562256157830336031652518559744 - (67682029681889335677290557259385*sin(q3L)*((16506520352940097956833727997725*cos(q2L))/20282409603651670423947251286016 + (7514214926474921*cos(q2L)*((1888752292310023*cos(q1L))/18014398509481984 - (5148155107303929*sin(q1L))/9007199254740992))/36893488147419103232 + sin(q2L)*((5148155107303929*cos(q1L))/9007199254740992 + (1888752292310023*sin(q1L))/18014398509481984)))/332306998946228968225951765070086144 + (508577317689771495245073589786522929324694383585*cos(q3L)*((16506520352940097956833727997725*sin(q2L))/20282409603651670423947251286016 - cos(q2L)*((5148155107303929*cos(q1L))/9007199254740992 + (1888752292310023*sin(q1L))/18014398509481984) + (7514214926474921*sin(q2L)*((1888752292310023*cos(q1L))/18014398509481984 - (5148155107303929*sin(q1L))/9007199254740992))/36893488147419103232))/12259964326927110866866776217202473468949912977468817408 - (13258697167433729449897784796786197386719169465*sin(q3L)*((16506520352940097956833727997725*sin(q2L))/20282409603651670423947251286016 - cos(q2L)*((5148155107303929*cos(q1L))/9007199254740992 + (1888752292310023*sin(q1L))/18014398509481984) + (7514214926474921*sin(q2L)*((1888752292310023*cos(q1L))/18014398509481984 - (5148155107303929*sin(q1L))/9007199254740992))/36893488147419103232))/1569275433846670190958947355801916604025588861116008628224))/1801439850948198400 - (60617164743372705924380750591060836759586313939367162716784907429017787816377231*cos(q3L)*((16506520352940097956833727997725*cos(q2L))/20282409603651670423947251286016 + (7514214926474921*cos(q2L)*((1888752292310023*cos(q1L))/18014398509481984 - (5148155107303929*sin(q1L))/9007199254740992))/36893488147419103232 + sin(q2L)*((5148155107303929*cos(q1L))/9007199254740992 + (1888752292310023*sin(q1L))/18014398509481984)))/1447401115466452442794637312608598848165874808320507050493219800098914120499200000 - (3*sin(q2L)*((5148155107303929*cos(q1L))/9007199254740992 + (1888752292310023*sin(q1L))/18014398509481984))/100 - (807520961047489018778067709720399904923771262077295170375712179706208528987338271217011451790113918662491539890779991*sin(q2L)*((1888752292310023*cos(q1L))/18014398509481984 - (5148155107303929*sin(q1L))/9007199254740992))/15760802478557791684911616040057445522031895708186178667179317361698288708598884244565706501953966256322651196122726400000 + (608651409044468601*sin(q4L)*(sin(q3L)*((16506520352940097956833727997725*cos(q2L))/20282409603651670423947251286016 + (7514214926474921*cos(q2L)*((1888752292310023*cos(q1L))/18014398509481984 - (5148155107303929*sin(q1L))/9007199254740992))/36893488147419103232 + sin(q2L)*((5148155107303929*cos(q1L))/9007199254740992 + (1888752292310023*sin(q1L))/18014398509481984)) - (7514214926474921*cos(q3L)*((16506520352940097956833727997725*sin(q2L))/20282409603651670423947251286016 - cos(q2L)*((5148155107303929*cos(q1L))/9007199254740992 + (1888752292310023*sin(q1L))/18014398509481984) + (7514214926474921*sin(q2L)*((1888752292310023*cos(q1L))/18014398509481984 - (5148155107303929*sin(q1L))/9007199254740992))/36893488147419103232))/36893488147419103232))/73786976294838206464000 + (94754841554645069948206780163139*sin(q5L)*(((7514214926474921*cos(q4L))/36893488147419103232 + (4503599440548691*sin(q4L))/4503599627370496)*(cos(q3L)*((16506520352940097956833727997725*cos(q2L))/20282409603651670423947251286016 + (7514214926474921*cos(q2L)*((1888752292310023*cos(q1L))/18014398509481984 - (5148155107303929*sin(q1L))/9007199254740992))/36893488147419103232 + sin(q2L)*((5148155107303929*cos(q1L))/9007199254740992 + (1888752292310023*sin(q1L))/18014398509481984)) + (7514214926474921*sin(q3L)*((16506520352940097956833727997725*sin(q2L))/20282409603651670423947251286016 - cos(q2L)*((5148155107303929*cos(q1L))/9007199254740992 + (1888752292310023*sin(q1L))/18014398509481984) + (7514214926474921*sin(q2L)*((1888752292310023*cos(q1L))/18014398509481984 - (5148155107303929*sin(q1L))/9007199254740992))/36893488147419103232))/36893488147419103232) + ((9007199067919185*cos(q4L))/9007199254740992 - (234819211581865*sin(q4L))/1152921504606846976)*((148677514737591106934298605035692608392163854125*sin(q2L))/182687704666362864775460604089535377456991567872 - (9007199067919185*cos(q2L)*((5148155107303929*cos(q1L))/9007199254740992 + (1888752292310023*sin(q1L))/18014398509481984))/9007199254740992 + (67682029681889335677290557259385*sin(q2L)*((1888752292310023*cos(q1L))/18014398509481984 - (5148155107303929*sin(q1L))/9007199254740992))/332306998946228968225951765070086144) - (7514214926474921*sin(q4L)*(sin(q3L)*((16506520352940097956833727997725*cos(q2L))/20282409603651670423947251286016 + (7514214926474921*cos(q2L)*((1888752292310023*cos(q1L))/18014398509481984 - (5148155107303929*sin(q1L))/9007199254740992))/36893488147419103232 + sin(q2L)*((5148155107303929*cos(q1L))/9007199254740992 + (1888752292310023*sin(q1L))/18014398509481984)) - (7514214926474921*cos(q3L)*((16506520352940097956833727997725*sin(q2L))/20282409603651670423947251286016 - cos(q2L)*((5148155107303929*cos(q1L))/9007199254740992 + (1888752292310023*sin(q1L))/18014398509481984) + (7514214926474921*sin(q2L)*((1888752292310023*cos(q1L))/18014398509481984 - (5148155107303929*sin(q1L))/9007199254740992))/36893488147419103232))/36893488147419103232))/36893488147419103232))/66461399789245793645190353014017228800 - (27*cos(q6L)*((9007199067919185*sin(q5L)*((14115856197532180673579726082375*cos(q2L)*((5148155107303929*cos(q1L))/9007199254740992 + (1888752292310023*sin(q1L))/18014398509481984))/340282366920938463463374607431768211456 - (233003667623740560033643537092505706768317191960312467162596875*sin(q2L))/6901746346790563787434755862277025452451108972170386555162524223799296 + (234819211581865*cos(q3L)*((16506520352940097956833727997725*cos(q2L))/20282409603651670423947251286016 + (7514214926474921*cos(q2L)*((1888752292310023*cos(q1L))/18014398509481984 - (5148155107303929*sin(q1L))/9007199254740992))/36893488147419103232 + sin(q2L)*((5148155107303929*cos(q1L))/9007199254740992 + (1888752292310023*sin(q1L))/18014398509481984)))/1152921504606846976 - (106069577339469832923929692356850887620017617375*sin(q2L)*((1888752292310023*cos(q1L))/18014398509481984 - (5148155107303929*sin(q1L))/9007199254740992))/12554203470773361527671578846415332832204710888928069025792 + (9007199067919185*sin(q3L)*((16506520352940097956833727997725*cos(q2L))/20282409603651670423947251286016 + (7514214926474921*cos(q2L)*((1888752292310023*cos(q1L))/18014398509481984 - (5148155107303929*sin(q1L))/9007199254740992))/36893488147419103232 + sin(q2L)*((5148155107303929*cos(q1L))/9007199254740992 + (1888752292310023*sin(q1L))/18014398509481984)))/9007199254740992 - (67682029681889335677290557259385*cos(q3L)*((16506520352940097956833727997725*sin(q2L))/20282409603651670423947251286016 - cos(q2L)*((5148155107303929*cos(q1L))/9007199254740992 + (1888752292310023*sin(q1L))/18014398509481984) + (7514214926474921*sin(q2L)*((1888752292310023*cos(q1L))/18014398509481984 - (5148155107303929*sin(q1L))/9007199254740992))/36893488147419103232))/332306998946228968225951765070086144 + (1764482024691522628700660907665*sin(q3L)*((16506520352940097956833727997725*sin(q2L))/20282409603651670423947251286016 - cos(q2L)*((5148155107303929*cos(q1L))/9007199254740992 + (1888752292310023*sin(q1L))/18014398509481984) + (7514214926474921*sin(q2L)*((1888752292310023*cos(q1L))/18014398509481984 - (5148155107303929*sin(q1L))/9007199254740992))/36893488147419103232))/42535295865117307932921825928971026432))/9007199254740992 + cos(q5L)*(((7514214926474921*cos(q4L))/36893488147419103232 + (4503599440548691*sin(q4L))/4503599627370496)*(cos(q3L)*((16506520352940097956833727997725*cos(q2L))/20282409603651670423947251286016 + (7514214926474921*cos(q2L)*((1888752292310023*cos(q1L))/18014398509481984 - (5148155107303929*sin(q1L))/9007199254740992))/36893488147419103232 + sin(q2L)*((5148155107303929*cos(q1L))/9007199254740992 + (1888752292310023*sin(q1L))/18014398509481984)) + (7514214926474921*sin(q3L)*((16506520352940097956833727997725*sin(q2L))/20282409603651670423947251286016 - cos(q2L)*((5148155107303929*cos(q1L))/9007199254740992 + (1888752292310023*sin(q1L))/18014398509481984) + (7514214926474921*sin(q2L)*((1888752292310023*cos(q1L))/18014398509481984 - (5148155107303929*sin(q1L))/9007199254740992))/36893488147419103232))/36893488147419103232) + ((9007199067919185*cos(q4L))/9007199254740992 - (234819211581865*sin(q4L))/1152921504606846976)*((148677514737591106934298605035692608392163854125*sin(q2L))/182687704666362864775460604089535377456991567872 - (9007199067919185*cos(q2L)*((5148155107303929*cos(q1L))/9007199254740992 + (1888752292310023*sin(q1L))/18014398509481984))/9007199254740992 + (67682029681889335677290557259385*sin(q2L)*((1888752292310023*cos(q1L))/18014398509481984 - (5148155107303929*sin(q1L))/9007199254740992))/332306998946228968225951765070086144) - (7514214926474921*sin(q4L)*(sin(q3L)*((16506520352940097956833727997725*cos(q2L))/20282409603651670423947251286016 + (7514214926474921*cos(q2L)*((1888752292310023*cos(q1L))/18014398509481984 - (5148155107303929*sin(q1L))/9007199254740992))/36893488147419103232 + sin(q2L)*((5148155107303929*cos(q1L))/9007199254740992 + (1888752292310023*sin(q1L))/18014398509481984)) - (7514214926474921*cos(q3L)*((16506520352940097956833727997725*sin(q2L))/20282409603651670423947251286016 - cos(q2L)*((5148155107303929*cos(q1L))/9007199254740992 + (1888752292310023*sin(q1L))/18014398509481984) + (7514214926474921*sin(q2L)*((1888752292310023*cos(q1L))/18014398509481984 - (5148155107303929*sin(q1L))/9007199254740992))/36893488147419103232))/36893488147419103232))/36893488147419103232) + (7514214926474921*sin(q5L)*(((234819211581865*cos(q4L))/1152921504606846976 + (9007199067919185*sin(q4L))/9007199254740992)*((148677514737591106934298605035692608392163854125*sin(q2L))/182687704666362864775460604089535377456991567872 - (9007199067919185*cos(q2L)*((5148155107303929*cos(q1L))/9007199254740992 + (1888752292310023*sin(q1L))/18014398509481984))/9007199254740992 + (67682029681889335677290557259385*sin(q2L)*((1888752292310023*cos(q1L))/18014398509481984 - (5148155107303929*sin(q1L))/9007199254740992))/332306998946228968225951765070086144) - ((4503599440548691*cos(q4L))/4503599627370496 - (7514214926474921*sin(q4L))/36893488147419103232)*(cos(q3L)*((16506520352940097956833727997725*cos(q2L))/20282409603651670423947251286016 + (7514214926474921*cos(q2L)*((1888752292310023*cos(q1L))/18014398509481984 - (5148155107303929*sin(q1L))/9007199254740992))/36893488147419103232 + sin(q2L)*((5148155107303929*cos(q1L))/9007199254740992 + (1888752292310023*sin(q1L))/18014398509481984)) + (7514214926474921*sin(q3L)*((16506520352940097956833727997725*sin(q2L))/20282409603651670423947251286016 - cos(q2L)*((5148155107303929*cos(q1L))/9007199254740992 + (1888752292310023*sin(q1L))/18014398509481984) + (7514214926474921*sin(q2L)*((1888752292310023*cos(q1L))/18014398509481984 - (5148155107303929*sin(q1L))/9007199254740992))/36893488147419103232))/36893488147419103232) + (7514214926474921*cos(q4L)*(sin(q3L)*((16506520352940097956833727997725*cos(q2L))/20282409603651670423947251286016 + (7514214926474921*cos(q2L)*((1888752292310023*cos(q1L))/18014398509481984 - (5148155107303929*sin(q1L))/9007199254740992))/36893488147419103232 + sin(q2L)*((5148155107303929*cos(q1L))/9007199254740992 + (1888752292310023*sin(q1L))/18014398509481984)) - (7514214926474921*cos(q3L)*((16506520352940097956833727997725*sin(q2L))/20282409603651670423947251286016 - cos(q2L)*((5148155107303929*cos(q1L))/9007199254740992 + (1888752292310023*sin(q1L))/18014398509481984) + (7514214926474921*sin(q2L)*((1888752292310023*cos(q1L))/18014398509481984 - (5148155107303929*sin(q1L))/9007199254740992))/36893488147419103232))/36893488147419103232))/36893488147419103232))/36893488147419103232))/1000 + (202883803014822867*sin(q6L)*((9007199067919185*cos(q5L)*((14115856197532180673579726082375*cos(q2L)*((5148155107303929*cos(q1L))/9007199254740992 + (1888752292310023*sin(q1L))/18014398509481984))/340282366920938463463374607431768211456 - (233003667623740560033643537092505706768317191960312467162596875*sin(q2L))/6901746346790563787434755862277025452451108972170386555162524223799296 + (234819211581865*cos(q3L)*((16506520352940097956833727997725*cos(q2L))/20282409603651670423947251286016 + (7514214926474921*cos(q2L)*((1888752292310023*cos(q1L))/18014398509481984 - (5148155107303929*sin(q1L))/9007199254740992))/36893488147419103232 + sin(q2L)*((5148155107303929*cos(q1L))/9007199254740992 + (1888752292310023*sin(q1L))/18014398509481984)))/1152921504606846976 - (106069577339469832923929692356850887620017617375*sin(q2L)*((1888752292310023*cos(q1L))/18014398509481984 - (5148155107303929*sin(q1L))/9007199254740992))/12554203470773361527671578846415332832204710888928069025792 + (9007199067919185*sin(q3L)*((16506520352940097956833727997725*cos(q2L))/20282409603651670423947251286016 + (7514214926474921*cos(q2L)*((1888752292310023*cos(q1L))/18014398509481984 - (5148155107303929*sin(q1L))/9007199254740992))/36893488147419103232 + sin(q2L)*((5148155107303929*cos(q1L))/9007199254740992 + (1888752292310023*sin(q1L))/18014398509481984)))/9007199254740992 - (67682029681889335677290557259385*cos(q3L)*((16506520352940097956833727997725*sin(q2L))/20282409603651670423947251286016 - cos(q2L)*((5148155107303929*cos(q1L))/9007199254740992 + (1888752292310023*sin(q1L))/18014398509481984) + (7514214926474921*sin(q2L)*((1888752292310023*cos(q1L))/18014398509481984 - (5148155107303929*sin(q1L))/9007199254740992))/36893488147419103232))/332306998946228968225951765070086144 + (1764482024691522628700660907665*sin(q3L)*((16506520352940097956833727997725*sin(q2L))/20282409603651670423947251286016 - cos(q2L)*((5148155107303929*cos(q1L))/9007199254740992 + (1888752292310023*sin(q1L))/18014398509481984) + (7514214926474921*sin(q2L)*((1888752292310023*cos(q1L))/18014398509481984 - (5148155107303929*sin(q1L))/9007199254740992))/36893488147419103232))/42535295865117307932921825928971026432))/9007199254740992 + (7514214926474921*cos(q5L)*(((234819211581865*cos(q4L))/1152921504606846976 + (9007199067919185*sin(q4L))/9007199254740992)*((148677514737591106934298605035692608392163854125*sin(q2L))/182687704666362864775460604089535377456991567872 - (9007199067919185*cos(q2L)*((5148155107303929*cos(q1L))/9007199254740992 + (1888752292310023*sin(q1L))/18014398509481984))/9007199254740992 + (67682029681889335677290557259385*sin(q2L)*((1888752292310023*cos(q1L))/18014398509481984 - (5148155107303929*sin(q1L))/9007199254740992))/332306998946228968225951765070086144) - ((4503599440548691*cos(q4L))/4503599627370496 - (7514214926474921*sin(q4L))/36893488147419103232)*(cos(q3L)*((16506520352940097956833727997725*cos(q2L))/20282409603651670423947251286016 + (7514214926474921*cos(q2L)*((1888752292310023*cos(q1L))/18014398509481984 - (5148155107303929*sin(q1L))/9007199254740992))/36893488147419103232 + sin(q2L)*((5148155107303929*cos(q1L))/9007199254740992 + (1888752292310023*sin(q1L))/18014398509481984)) + (7514214926474921*sin(q3L)*((16506520352940097956833727997725*sin(q2L))/20282409603651670423947251286016 - cos(q2L)*((5148155107303929*cos(q1L))/9007199254740992 + (1888752292310023*sin(q1L))/18014398509481984) + (7514214926474921*sin(q2L)*((1888752292310023*cos(q1L))/18014398509481984 - (5148155107303929*sin(q1L))/9007199254740992))/36893488147419103232))/36893488147419103232) + (7514214926474921*cos(q4L)*(sin(q3L)*((16506520352940097956833727997725*cos(q2L))/20282409603651670423947251286016 + (7514214926474921*cos(q2L)*((1888752292310023*cos(q1L))/18014398509481984 - (5148155107303929*sin(q1L))/9007199254740992))/36893488147419103232 + sin(q2L)*((5148155107303929*cos(q1L))/9007199254740992 + (1888752292310023*sin(q1L))/18014398509481984)) - (7514214926474921*cos(q3L)*((16506520352940097956833727997725*sin(q2L))/20282409603651670423947251286016 - cos(q2L)*((5148155107303929*cos(q1L))/9007199254740992 + (1888752292310023*sin(q1L))/18014398509481984) + (7514214926474921*sin(q2L)*((1888752292310023*cos(q1L))/18014398509481984 - (5148155107303929*sin(q1L))/9007199254740992))/36893488147419103232))/36893488147419103232))/36893488147419103232))/36893488147419103232 - sin(q5L)*(((7514214926474921*cos(q4L))/36893488147419103232 + (4503599440548691*sin(q4L))/4503599627370496)*(cos(q3L)*((16506520352940097956833727997725*cos(q2L))/20282409603651670423947251286016 + (7514214926474921*cos(q2L)*((1888752292310023*cos(q1L))/18014398509481984 - (5148155107303929*sin(q1L))/9007199254740992))/36893488147419103232 + sin(q2L)*((5148155107303929*cos(q1L))/9007199254740992 + (1888752292310023*sin(q1L))/18014398509481984)) + (7514214926474921*sin(q3L)*((16506520352940097956833727997725*sin(q2L))/20282409603651670423947251286016 - cos(q2L)*((5148155107303929*cos(q1L))/9007199254740992 + (1888752292310023*sin(q1L))/18014398509481984) + (7514214926474921*sin(q2L)*((1888752292310023*cos(q1L))/18014398509481984 - (5148155107303929*sin(q1L))/9007199254740992))/36893488147419103232))/36893488147419103232) + ((9007199067919185*cos(q4L))/9007199254740992 - (234819211581865*sin(q4L))/1152921504606846976)*((148677514737591106934298605035692608392163854125*sin(q2L))/182687704666362864775460604089535377456991567872 - (9007199067919185*cos(q2L)*((5148155107303929*cos(q1L))/9007199254740992 + (1888752292310023*sin(q1L))/18014398509481984))/9007199254740992 + (67682029681889335677290557259385*sin(q2L)*((1888752292310023*cos(q1L))/18014398509481984 - (5148155107303929*sin(q1L))/9007199254740992))/332306998946228968225951765070086144) - (7514214926474921*sin(q4L)*(sin(q3L)*((16506520352940097956833727997725*cos(q2L))/20282409603651670423947251286016 + (7514214926474921*cos(q2L)*((1888752292310023*cos(q1L))/18014398509481984 - (5148155107303929*sin(q1L))/9007199254740992))/36893488147419103232 + sin(q2L)*((5148155107303929*cos(q1L))/9007199254740992 + (1888752292310023*sin(q1L))/18014398509481984)) - (7514214926474921*cos(q3L)*((16506520352940097956833727997725*sin(q2L))/20282409603651670423947251286016 - cos(q2L)*((5148155107303929*cos(q1L))/9007199254740992 + (1888752292310023*sin(q1L))/18014398509481984) + (7514214926474921*sin(q2L)*((1888752292310023*cos(q1L))/18014398509481984 - (5148155107303929*sin(q1L))/9007199254740992))/36893488147419103232))/36893488147419103232))/36893488147419103232)))/36893488147419103232000 - (46241644459901303158631016767207157814229090534989303509431886332469146043*sin(q3L)*((16506520352940097956833727997725*cos(q2L))/20282409603651670423947251286016 + (7514214926474921*cos(q2L)*((1888752292310023*cos(q1L))/18014398509481984 - (5148155107303929*sin(q1L))/9007199254740992))/36893488147419103232 + sin(q2L)*((5148155107303929*cos(q1L))/9007199254740992 + (1888752292310023*sin(q1L))/18014398509481984)))/2261564242916331941866620800950935700259179388000792266395655937654553313280000 + (347469655025336708709976918716104493695816557877713443586884917071777956519687017125887603*cos(q3L)*((16506520352940097956833727997725*sin(q2L))/20282409603651670423947251286016 - cos(q2L)*((5148155107303929*cos(q1L))/9007199254740992 + (1888752292310023*sin(q1L))/18014398509481984) + (7514214926474921*sin(q2L)*((1888752292310023*cos(q1L))/18014398509481984 - (5148155107303929*sin(q1L))/9007199254740992))/36893488147419103232))/83436993590660550093555535397248129476668145404556748826056312805555458038306271485271956520960000 + (324259171862923063*sin(q6L)*((9007199067919185*sin(q5L)*((14115856197532180673579726082375*cos(q2L)*((5148155107303929*cos(q1L))/9007199254740992 + (1888752292310023*sin(q1L))/18014398509481984))/340282366920938463463374607431768211456 - (233003667623740560033643537092505706768317191960312467162596875*sin(q2L))/6901746346790563787434755862277025452451108972170386555162524223799296 + (234819211581865*cos(q3L)*((16506520352940097956833727997725*cos(q2L))/20282409603651670423947251286016 + (7514214926474921*cos(q2L)*((1888752292310023*cos(q1L))/18014398509481984 - (5148155107303929*sin(q1L))/9007199254740992))/36893488147419103232 + sin(q2L)*((5148155107303929*cos(q1L))/9007199254740992 + (1888752292310023*sin(q1L))/18014398509481984)))/1152921504606846976 - (106069577339469832923929692356850887620017617375*sin(q2L)*((1888752292310023*cos(q1L))/18014398509481984 - (5148155107303929*sin(q1L))/9007199254740992))/12554203470773361527671578846415332832204710888928069025792 + (9007199067919185*sin(q3L)*((16506520352940097956833727997725*cos(q2L))/20282409603651670423947251286016 + (7514214926474921*cos(q2L)*((1888752292310023*cos(q1L))/18014398509481984 - (5148155107303929*sin(q1L))/9007199254740992))/36893488147419103232 + sin(q2L)*((5148155107303929*cos(q1L))/9007199254740992 + (1888752292310023*sin(q1L))/18014398509481984)))/9007199254740992 - (67682029681889335677290557259385*cos(q3L)*((16506520352940097956833727997725*sin(q2L))/20282409603651670423947251286016 - cos(q2L)*((5148155107303929*cos(q1L))/9007199254740992 + (1888752292310023*sin(q1L))/18014398509481984) + (7514214926474921*sin(q2L)*((1888752292310023*cos(q1L))/18014398509481984 - (5148155107303929*sin(q1L))/9007199254740992))/36893488147419103232))/332306998946228968225951765070086144 + (1764482024691522628700660907665*sin(q3L)*((16506520352940097956833727997725*sin(q2L))/20282409603651670423947251286016 - cos(q2L)*((5148155107303929*cos(q1L))/9007199254740992 + (1888752292310023*sin(q1L))/18014398509481984) + (7514214926474921*sin(q2L)*((1888752292310023*cos(q1L))/18014398509481984 - (5148155107303929*sin(q1L))/9007199254740992))/36893488147419103232))/42535295865117307932921825928971026432))/9007199254740992 + cos(q5L)*(((7514214926474921*cos(q4L))/36893488147419103232 + (4503599440548691*sin(q4L))/4503599627370496)*(cos(q3L)*((16506520352940097956833727997725*cos(q2L))/20282409603651670423947251286016 + (7514214926474921*cos(q2L)*((1888752292310023*cos(q1L))/18014398509481984 - (5148155107303929*sin(q1L))/9007199254740992))/36893488147419103232 + sin(q2L)*((5148155107303929*cos(q1L))/9007199254740992 + (1888752292310023*sin(q1L))/18014398509481984)) + (7514214926474921*sin(q3L)*((16506520352940097956833727997725*sin(q2L))/20282409603651670423947251286016 - cos(q2L)*((5148155107303929*cos(q1L))/9007199254740992 + (1888752292310023*sin(q1L))/18014398509481984) + (7514214926474921*sin(q2L)*((1888752292310023*cos(q1L))/18014398509481984 - (5148155107303929*sin(q1L))/9007199254740992))/36893488147419103232))/36893488147419103232) + ((9007199067919185*cos(q4L))/9007199254740992 - (234819211581865*sin(q4L))/1152921504606846976)*((148677514737591106934298605035692608392163854125*sin(q2L))/182687704666362864775460604089535377456991567872 - (9007199067919185*cos(q2L)*((5148155107303929*cos(q1L))/9007199254740992 + (1888752292310023*sin(q1L))/18014398509481984))/9007199254740992 + (67682029681889335677290557259385*sin(q2L)*((1888752292310023*cos(q1L))/18014398509481984 - (5148155107303929*sin(q1L))/9007199254740992))/332306998946228968225951765070086144) - (7514214926474921*sin(q4L)*(sin(q3L)*((16506520352940097956833727997725*cos(q2L))/20282409603651670423947251286016 + (7514214926474921*cos(q2L)*((1888752292310023*cos(q1L))/18014398509481984 - (5148155107303929*sin(q1L))/9007199254740992))/36893488147419103232 + sin(q2L)*((5148155107303929*cos(q1L))/9007199254740992 + (1888752292310023*sin(q1L))/18014398509481984)) - (7514214926474921*cos(q3L)*((16506520352940097956833727997725*sin(q2L))/20282409603651670423947251286016 - cos(q2L)*((5148155107303929*cos(q1L))/9007199254740992 + (1888752292310023*sin(q1L))/18014398509481984) + (7514214926474921*sin(q2L)*((1888752292310023*cos(q1L))/18014398509481984 - (5148155107303929*sin(q1L))/9007199254740992))/36893488147419103232))/36893488147419103232))/36893488147419103232) + (7514214926474921*sin(q5L)*(((234819211581865*cos(q4L))/1152921504606846976 + (9007199067919185*sin(q4L))/9007199254740992)*((148677514737591106934298605035692608392163854125*sin(q2L))/182687704666362864775460604089535377456991567872 - (9007199067919185*cos(q2L)*((5148155107303929*cos(q1L))/9007199254740992 + (1888752292310023*sin(q1L))/18014398509481984))/9007199254740992 + (67682029681889335677290557259385*sin(q2L)*((1888752292310023*cos(q1L))/18014398509481984 - (5148155107303929*sin(q1L))/9007199254740992))/332306998946228968225951765070086144) - ((4503599440548691*cos(q4L))/4503599627370496 - (7514214926474921*sin(q4L))/36893488147419103232)*(cos(q3L)*((16506520352940097956833727997725*cos(q2L))/20282409603651670423947251286016 + (7514214926474921*cos(q2L)*((1888752292310023*cos(q1L))/18014398509481984 - (5148155107303929*sin(q1L))/9007199254740992))/36893488147419103232 + sin(q2L)*((5148155107303929*cos(q1L))/9007199254740992 + (1888752292310023*sin(q1L))/18014398509481984)) + (7514214926474921*sin(q3L)*((16506520352940097956833727997725*sin(q2L))/20282409603651670423947251286016 - cos(q2L)*((5148155107303929*cos(q1L))/9007199254740992 + (1888752292310023*sin(q1L))/18014398509481984) + (7514214926474921*sin(q2L)*((1888752292310023*cos(q1L))/18014398509481984 - (5148155107303929*sin(q1L))/9007199254740992))/36893488147419103232))/36893488147419103232) + (7514214926474921*cos(q4L)*(sin(q3L)*((16506520352940097956833727997725*cos(q2L))/20282409603651670423947251286016 + (7514214926474921*cos(q2L)*((1888752292310023*cos(q1L))/18014398509481984 - (5148155107303929*sin(q1L))/9007199254740992))/36893488147419103232 + sin(q2L)*((5148155107303929*cos(q1L))/9007199254740992 + (1888752292310023*sin(q1L))/18014398509481984)) - (7514214926474921*cos(q3L)*((16506520352940097956833727997725*sin(q2L))/20282409603651670423947251286016 - cos(q2L)*((5148155107303929*cos(q1L))/9007199254740992 + (1888752292310023*sin(q1L))/18014398509481984) + (7514214926474921*sin(q2L)*((1888752292310023*cos(q1L))/18014398509481984 - (5148155107303929*sin(q1L))/9007199254740992))/36893488147419103232))/36893488147419103232))/36893488147419103232))/36893488147419103232))/9007199254740992000 - (455490404115240510935077772268745492204390157443214084883134054419271951750419293234291596923751*sin(q3L)*((16506520352940097956833727997725*sin(q2L))/20282409603651670423947251286016 - cos(q2L)*((5148155107303929*cos(q1L))/9007199254740992 + (1888752292310023*sin(q1L))/18014398509481984) + (7514214926474921*sin(q2L)*((1888752292310023*cos(q1L))/18014398509481984 - (5148155107303929*sin(q1L))/9007199254740992))/36893488147419103232))/53399675898022752059875542654238802865067613058916319248676040195555493144516013750574052173414400000, (202883803014822867*sin(q5L)*(((4503599440548691*cos(q4L))/4503599627370496 - (7514214926474921*sin(q4L))/36893488147419103232)*((7514214926474921*cos(q3L)*((16506520352940097956833727997725*cos(q2L))/20282409603651670423947251286016 + (7514214926474921*cos(q2L)*((1888752292310023*cos(q1L))/18014398509481984 - (5148155107303929*sin(q1L))/9007199254740992))/36893488147419103232 + sin(q2L)*((5148155107303929*cos(q1L))/9007199254740992 + (1888752292310023*sin(q1L))/18014398509481984)))/36893488147419103232 - (9007199067919185*cos(q3L)*((46370457884011341126541404977865*sin(q1L))/81129638414606681695789005144064 - (17012367886825063216155529491255*cos(q1L))/162259276829213363391578010288128 + 13770489658876653055167369550485/83076749736557242056487941267521536))/9007199254740992 + sin(q3L)*((16506520352940097956833727997725*sin(q2L))/20282409603651670423947251286016 - cos(q2L)*((5148155107303929*cos(q1L))/9007199254740992 + (1888752292310023*sin(q1L))/18014398509481984) + (7514214926474921*sin(q2L)*((1888752292310023*cos(q1L))/18014398509481984 - (5148155107303929*sin(q1L))/9007199254740992))/36893488147419103232)) + (7514214926474921*cos(q4L)*((9007199067919185*sin(q3L)*((46370457884011341126541404977865*sin(q1L))/81129638414606681695789005144064 - (17012367886825063216155529491255*cos(q1L))/162259276829213363391578010288128 + 13770489658876653055167369550485/83076749736557242056487941267521536))/9007199254740992 - (7514214926474921*sin(q3L)*((16506520352940097956833727997725*cos(q2L))/20282409603651670423947251286016 + (7514214926474921*cos(q2L)*((1888752292310023*cos(q1L))/18014398509481984 - (5148155107303929*sin(q1L))/9007199254740992))/36893488147419103232 + sin(q2L)*((5148155107303929*cos(q1L))/9007199254740992 + (1888752292310023*sin(q1L))/18014398509481984)))/36893488147419103232 + cos(q3L)*((16506520352940097956833727997725*sin(q2L))/20282409603651670423947251286016 - cos(q2L)*((5148155107303929*cos(q1L))/9007199254740992 + (1888752292310023*sin(q1L))/18014398509481984) + (7514214926474921*sin(q2L)*((1888752292310023*cos(q1L))/18014398509481984 - (5148155107303929*sin(q1L))/9007199254740992))/36893488147419103232)))/36893488147419103232))/36893488147419103232000 - (712008244765680093343103025701132101054572137019*cos(q5L)*(((4503599440548691*cos(q4L))/4503599627370496 - (7514214926474921*sin(q4L))/36893488147419103232)*((7514214926474921*cos(q3L)*((16506520352940097956833727997725*cos(q2L))/20282409603651670423947251286016 + (7514214926474921*cos(q2L)*((1888752292310023*cos(q1L))/18014398509481984 - (5148155107303929*sin(q1L))/9007199254740992))/36893488147419103232 + sin(q2L)*((5148155107303929*cos(q1L))/9007199254740992 + (1888752292310023*sin(q1L))/18014398509481984)))/36893488147419103232 - (9007199067919185*cos(q3L)*((46370457884011341126541404977865*sin(q1L))/81129638414606681695789005144064 - (17012367886825063216155529491255*cos(q1L))/162259276829213363391578010288128 + 13770489658876653055167369550485/83076749736557242056487941267521536))/9007199254740992 + sin(q3L)*((16506520352940097956833727997725*sin(q2L))/20282409603651670423947251286016 - cos(q2L)*((5148155107303929*cos(q1L))/9007199254740992 + (1888752292310023*sin(q1L))/18014398509481984) + (7514214926474921*sin(q2L)*((1888752292310023*cos(q1L))/18014398509481984 - (5148155107303929*sin(q1L))/9007199254740992))/36893488147419103232)) + (7514214926474921*cos(q4L)*((9007199067919185*sin(q3L)*((46370457884011341126541404977865*sin(q1L))/81129638414606681695789005144064 - (17012367886825063216155529491255*cos(q1L))/162259276829213363391578010288128 + 13770489658876653055167369550485/83076749736557242056487941267521536))/9007199254740992 - (7514214926474921*sin(q3L)*((16506520352940097956833727997725*cos(q2L))/20282409603651670423947251286016 + (7514214926474921*cos(q2L)*((1888752292310023*cos(q1L))/18014398509481984 - (5148155107303929*sin(q1L))/9007199254740992))/36893488147419103232 + sin(q2L)*((5148155107303929*cos(q1L))/9007199254740992 + (1888752292310023*sin(q1L))/18014398509481984)))/36893488147419103232 + cos(q3L)*((16506520352940097956833727997725*sin(q2L))/20282409603651670423947251286016 - cos(q2L)*((5148155107303929*cos(q1L))/9007199254740992 + (1888752292310023*sin(q1L))/18014398509481984) + (7514214926474921*sin(q2L)*((1888752292310023*cos(q1L))/18014398509481984 - (5148155107303929*sin(q1L))/9007199254740992))/36893488147419103232)))/36893488147419103232))/2451992865385422173373355243440494693789982595493763481600 - (83301539375654672537075965313343183841442266989297270401707771044036658496661398777306991*sin(q3L)*((46370457884011341126541404977865*sin(q1L))/81129638414606681695789005144064 - (17012367886825063216155529491255*cos(q1L))/162259276829213363391578010288128 + 13770489658876653055167369550485/83076749736557242056487941267521536))/4074071952668972172536891376818756322102936787331872501272280898708762599526673412366794752000 - (27*cos(q5L)*(((7514214926474921*cos(q4L))/36893488147419103232 + (4503599440548691*sin(q4L))/4503599627370496)*((7514214926474921*cos(q3L)*((16506520352940097956833727997725*cos(q2L))/20282409603651670423947251286016 + (7514214926474921*cos(q2L)*((1888752292310023*cos(q1L))/18014398509481984 - (5148155107303929*sin(q1L))/9007199254740992))/36893488147419103232 + sin(q2L)*((5148155107303929*cos(q1L))/9007199254740992 + (1888752292310023*sin(q1L))/18014398509481984)))/36893488147419103232 - (9007199067919185*cos(q3L)*((46370457884011341126541404977865*sin(q1L))/81129638414606681695789005144064 - (17012367886825063216155529491255*cos(q1L))/162259276829213363391578010288128 + 13770489658876653055167369550485/83076749736557242056487941267521536))/9007199254740992 + sin(q3L)*((16506520352940097956833727997725*sin(q2L))/20282409603651670423947251286016 - cos(q2L)*((5148155107303929*cos(q1L))/9007199254740992 + (1888752292310023*sin(q1L))/18014398509481984) + (7514214926474921*sin(q2L)*((1888752292310023*cos(q1L))/18014398509481984 - (5148155107303929*sin(q1L))/9007199254740992))/36893488147419103232)) + (7514214926474921*sin(q4L)*((9007199067919185*sin(q3L)*((46370457884011341126541404977865*sin(q1L))/81129638414606681695789005144064 - (17012367886825063216155529491255*cos(q1L))/162259276829213363391578010288128 + 13770489658876653055167369550485/83076749736557242056487941267521536))/9007199254740992 - (7514214926474921*sin(q3L)*((16506520352940097956833727997725*cos(q2L))/20282409603651670423947251286016 + (7514214926474921*cos(q2L)*((1888752292310023*cos(q1L))/18014398509481984 - (5148155107303929*sin(q1L))/9007199254740992))/36893488147419103232 + sin(q2L)*((5148155107303929*cos(q1L))/9007199254740992 + (1888752292310023*sin(q1L))/18014398509481984)))/36893488147419103232 + cos(q3L)*((16506520352940097956833727997725*sin(q2L))/20282409603651670423947251286016 - cos(q2L)*((5148155107303929*cos(q1L))/9007199254740992 + (1888752292310023*sin(q1L))/18014398509481984) + (7514214926474921*sin(q2L)*((1888752292310023*cos(q1L))/18014398509481984 - (5148155107303929*sin(q1L))/9007199254740992))/36893488147419103232)))/36893488147419103232))/1000 - (109198173955282063961996941994332957526645881091499469714283881779231664456243735535448036415347*cos(q3L)*((46370457884011341126541404977865*sin(q1L))/81129638414606681695789005144064 - (17012367886825063216155529491255*cos(q1L))/162259276829213363391578010288128 + 13770489658876653055167369550485/83076749736557242056487941267521536))/2607406049708142190423610481164004046145879543892398400814259775173608063697070983914748641280000 - (94754841554645069948206780163139*sin(q5L)*(((7514214926474921*cos(q4L))/36893488147419103232 + (4503599440548691*sin(q4L))/4503599627370496)*((7514214926474921*cos(q3L)*((16506520352940097956833727997725*cos(q2L))/20282409603651670423947251286016 + (7514214926474921*cos(q2L)*((1888752292310023*cos(q1L))/18014398509481984 - (5148155107303929*sin(q1L))/9007199254740992))/36893488147419103232 + sin(q2L)*((5148155107303929*cos(q1L))/9007199254740992 + (1888752292310023*sin(q1L))/18014398509481984)))/36893488147419103232 - (9007199067919185*cos(q3L)*((46370457884011341126541404977865*sin(q1L))/81129638414606681695789005144064 - (17012367886825063216155529491255*cos(q1L))/162259276829213363391578010288128 + 13770489658876653055167369550485/83076749736557242056487941267521536))/9007199254740992 + sin(q3L)*((16506520352940097956833727997725*sin(q2L))/20282409603651670423947251286016 - cos(q2L)*((5148155107303929*cos(q1L))/9007199254740992 + (1888752292310023*sin(q1L))/18014398509481984) + (7514214926474921*sin(q2L)*((1888752292310023*cos(q1L))/18014398509481984 - (5148155107303929*sin(q1L))/9007199254740992))/36893488147419103232)) + (7514214926474921*sin(q4L)*((9007199067919185*sin(q3L)*((46370457884011341126541404977865*sin(q1L))/81129638414606681695789005144064 - (17012367886825063216155529491255*cos(q1L))/162259276829213363391578010288128 + 13770489658876653055167369550485/83076749736557242056487941267521536))/9007199254740992 - (7514214926474921*sin(q3L)*((16506520352940097956833727997725*cos(q2L))/20282409603651670423947251286016 + (7514214926474921*cos(q2L)*((1888752292310023*cos(q1L))/18014398509481984 - (5148155107303929*sin(q1L))/9007199254740992))/36893488147419103232 + sin(q2L)*((5148155107303929*cos(q1L))/9007199254740992 + (1888752292310023*sin(q1L))/18014398509481984)))/36893488147419103232 + cos(q3L)*((16506520352940097956833727997725*sin(q2L))/20282409603651670423947251286016 - cos(q2L)*((5148155107303929*cos(q1L))/9007199254740992 + (1888752292310023*sin(q1L))/18014398509481984) + (7514214926474921*sin(q2L)*((1888752292310023*cos(q1L))/18014398509481984 - (5148155107303929*sin(q1L))/9007199254740992))/36893488147419103232)))/36893488147419103232))/66461399789245793645190353014017228800 + (81222263116692158804177042061221826384594597321566869716687*((4503599440548691*cos(q4L))/4503599627370496 - (7514214926474921*sin(q4L))/36893488147419103232)*((7514214926474921*cos(q3L)*((16506520352940097956833727997725*cos(q2L))/20282409603651670423947251286016 + (7514214926474921*cos(q2L)*((1888752292310023*cos(q1L))/18014398509481984 - (5148155107303929*sin(q1L))/9007199254740992))/36893488147419103232 + sin(q2L)*((5148155107303929*cos(q1L))/9007199254740992 + (1888752292310023*sin(q1L))/18014398509481984)))/36893488147419103232 - (9007199067919185*cos(q3L)*((46370457884011341126541404977865*sin(q1L))/81129638414606681695789005144064 - (17012367886825063216155529491255*cos(q1L))/162259276829213363391578010288128 + 13770489658876653055167369550485/83076749736557242056487941267521536))/9007199254740992 + sin(q3L)*((16506520352940097956833727997725*sin(q2L))/20282409603651670423947251286016 - cos(q2L)*((5148155107303929*cos(q1L))/9007199254740992 + (1888752292310023*sin(q1L))/18014398509481984) + (7514214926474921*sin(q2L)*((1888752292310023*cos(q1L))/18014398509481984 - (5148155107303929*sin(q1L))/9007199254740992))/36893488147419103232)))/306499108173177771671669405430061836723747824436720435200000 + (81*((7514214926474921*cos(q4L))/36893488147419103232 + (4503599440548691*sin(q4L))/4503599627370496)*((7514214926474921*cos(q3L)*((16506520352940097956833727997725*cos(q2L))/20282409603651670423947251286016 + (7514214926474921*cos(q2L)*((1888752292310023*cos(q1L))/18014398509481984 - (5148155107303929*sin(q1L))/9007199254740992))/36893488147419103232 + sin(q2L)*((5148155107303929*cos(q1L))/9007199254740992 + (1888752292310023*sin(q1L))/18014398509481984)))/36893488147419103232 - (9007199067919185*cos(q3L)*((46370457884011341126541404977865*sin(q1L))/81129638414606681695789005144064 - (17012367886825063216155529491255*cos(q1L))/162259276829213363391578010288128 + 13770489658876653055167369550485/83076749736557242056487941267521536))/9007199254740992 + sin(q3L)*((16506520352940097956833727997725*sin(q2L))/20282409603651670423947251286016 - cos(q2L)*((5148155107303929*cos(q1L))/9007199254740992 + (1888752292310023*sin(q1L))/18014398509481984) + (7514214926474921*sin(q2L)*((1888752292310023*cos(q1L))/18014398509481984 - (5148155107303929*sin(q1L))/9007199254740992))/36893488147419103232)))/2000 - (170695144106365826517608855445768431563113584343*cos(q5L)*((2115063383689692319117831580025*cos(q3L)*((46370457884011341126541404977865*sin(q1L))/81129638414606681695789005144064 - (17012367886825063216155529491255*cos(q1L))/162259276829213363391578010288128 + 13770489658876653055167369550485/83076749736557242056487941267521536))/10384593717069655257060992658440192 + (81129635049124235038645691064225*sin(q3L)*((46370457884011341126541404977865*sin(q1L))/81129638414606681695789005144064 - (17012367886825063216155529491255*cos(q1L))/162259276829213363391578010288128 + 13770489658876653055167369550485/83076749736557242056487941267521536))/81129638414606681695789005144064 - (1764482024691522628700660907665*cos(q3L)*((16506520352940097956833727997725*cos(q2L))/20282409603651670423947251286016 + (7514214926474921*cos(q2L)*((1888752292310023*cos(q1L))/18014398509481984 - (5148155107303929*sin(q1L))/9007199254740992))/36893488147419103232 + sin(q2L)*((5148155107303929*cos(q1L))/9007199254740992 + (1888752292310023*sin(q1L))/18014398509481984)))/42535295865117307932921825928971026432 - (67682029681889335677290557259385*sin(q3L)*((16506520352940097956833727997725*cos(q2L))/20282409603651670423947251286016 + (7514214926474921*cos(q2L)*((1888752292310023*cos(q1L))/18014398509481984 - (5148155107303929*sin(q1L))/9007199254740992))/36893488147419103232 + sin(q2L)*((5148155107303929*cos(q1L))/9007199254740992 + (1888752292310023*sin(q1L))/18014398509481984)))/332306998946228968225951765070086144 + (9007199067919185*cos(q3L)*((16506520352940097956833727997725*sin(q2L))/20282409603651670423947251286016 - cos(q2L)*((5148155107303929*cos(q1L))/9007199254740992 + (1888752292310023*sin(q1L))/18014398509481984) + (7514214926474921*sin(q2L)*((1888752292310023*cos(q1L))/18014398509481984 - (5148155107303929*sin(q1L))/9007199254740992))/36893488147419103232))/9007199254740992 - (234819211581865*sin(q3L)*((16506520352940097956833727997725*sin(q2L))/20282409603651670423947251286016 - cos(q2L)*((5148155107303929*cos(q1L))/9007199254740992 + (1888752292310023*sin(q1L))/18014398509481984) + (7514214926474921*sin(q2L)*((1888752292310023*cos(q1L))/18014398509481984 - (5148155107303929*sin(q1L))/9007199254740992))/36893488147419103232))/1152921504606846976))/119726214130147567059245861496117904970213993920593920 + (48638874966763599*sin(q5L)*((2115063383689692319117831580025*cos(q3L)*((46370457884011341126541404977865*sin(q1L))/81129638414606681695789005144064 - (17012367886825063216155529491255*cos(q1L))/162259276829213363391578010288128 + 13770489658876653055167369550485/83076749736557242056487941267521536))/10384593717069655257060992658440192 + (81129635049124235038645691064225*sin(q3L)*((46370457884011341126541404977865*sin(q1L))/81129638414606681695789005144064 - (17012367886825063216155529491255*cos(q1L))/162259276829213363391578010288128 + 13770489658876653055167369550485/83076749736557242056487941267521536))/81129638414606681695789005144064 - (1764482024691522628700660907665*cos(q3L)*((16506520352940097956833727997725*cos(q2L))/20282409603651670423947251286016 + (7514214926474921*cos(q2L)*((1888752292310023*cos(q1L))/18014398509481984 - (5148155107303929*sin(q1L))/9007199254740992))/36893488147419103232 + sin(q2L)*((5148155107303929*cos(q1L))/9007199254740992 + (1888752292310023*sin(q1L))/18014398509481984)))/42535295865117307932921825928971026432 - (67682029681889335677290557259385*sin(q3L)*((16506520352940097956833727997725*cos(q2L))/20282409603651670423947251286016 + (7514214926474921*cos(q2L)*((1888752292310023*cos(q1L))/18014398509481984 - (5148155107303929*sin(q1L))/9007199254740992))/36893488147419103232 + sin(q2L)*((5148155107303929*cos(q1L))/9007199254740992 + (1888752292310023*sin(q1L))/18014398509481984)))/332306998946228968225951765070086144 + (9007199067919185*cos(q3L)*((16506520352940097956833727997725*sin(q2L))/20282409603651670423947251286016 - cos(q2L)*((5148155107303929*cos(q1L))/9007199254740992 + (1888752292310023*sin(q1L))/18014398509481984) + (7514214926474921*sin(q2L)*((1888752292310023*cos(q1L))/18014398509481984 - (5148155107303929*sin(q1L))/9007199254740992))/36893488147419103232))/9007199254740992 - (234819211581865*sin(q3L)*((16506520352940097956833727997725*sin(q2L))/20282409603651670423947251286016 - cos(q2L)*((5148155107303929*cos(q1L))/9007199254740992 + (1888752292310023*sin(q1L))/18014398509481984) + (7514214926474921*sin(q2L)*((1888752292310023*cos(q1L))/18014398509481984 - (5148155107303929*sin(q1L))/9007199254740992))/36893488147419103232))/1152921504606846976))/1801439850948198400 + (584133382113593486367040631332731*cos(q6L)*((9007199067919185*((4503599440548691*cos(q4L))/4503599627370496 - (7514214926474921*sin(q4L))/36893488147419103232)*((7514214926474921*cos(q3L)*((16506520352940097956833727997725*cos(q2L))/20282409603651670423947251286016 + (7514214926474921*cos(q2L)*((1888752292310023*cos(q1L))/18014398509481984 - (5148155107303929*sin(q1L))/9007199254740992))/36893488147419103232 + sin(q2L)*((5148155107303929*cos(q1L))/9007199254740992 + (1888752292310023*sin(q1L))/18014398509481984)))/36893488147419103232 - (9007199067919185*cos(q3L)*((46370457884011341126541404977865*sin(q1L))/81129638414606681695789005144064 - (17012367886825063216155529491255*cos(q1L))/162259276829213363391578010288128 + 13770489658876653055167369550485/83076749736557242056487941267521536))/9007199254740992 + sin(q3L)*((16506520352940097956833727997725*sin(q2L))/20282409603651670423947251286016 - cos(q2L)*((5148155107303929*cos(q1L))/9007199254740992 + (1888752292310023*sin(q1L))/18014398509481984) + (7514214926474921*sin(q2L)*((1888752292310023*cos(q1L))/18014398509481984 - (5148155107303929*sin(q1L))/9007199254740992))/36893488147419103232)))/9007199254740992 - (609625514665592237562888769449172969868262801225*sin(q3L)*((46370457884011341126541404977865*sin(q1L))/81129638414606681695789005144064 - (17012367886825063216155529491255*cos(q1L))/162259276829213363391578010288128 + 13770489658876653055167369550485/83076749736557242056487941267521536))/2993155353253689176481146537402947624255349848014848 - (15893040848161638993908057577265778144967053025*cos(q3L)*((46370457884011341126541404977865*sin(q1L))/81129638414606681695789005144064 - (17012367886825063216155529491255*cos(q1L))/162259276829213363391578010288128 + 13770489658876653055167369550485/83076749736557242056487941267521536))/383123885216472214589586756787577295904684780545900544 + (13258697167433729449897784796786197386719169465*cos(q3L)*((16506520352940097956833727997725*cos(q2L))/20282409603651670423947251286016 + (7514214926474921*cos(q2L)*((1888752292310023*cos(q1L))/18014398509481984 - (5148155107303929*sin(q1L))/9007199254740992))/36893488147419103232 + sin(q2L)*((5148155107303929*cos(q1L))/9007199254740992 + (1888752292310023*sin(q1L))/18014398509481984)))/1569275433846670190958947355801916604025588861116008628224 + (67682029681889335677290557259385*cos(q4L)*((9007199067919185*sin(q3L)*((46370457884011341126541404977865*sin(q1L))/81129638414606681695789005144064 - (17012367886825063216155529491255*cos(q1L))/162259276829213363391578010288128 + 13770489658876653055167369550485/83076749736557242056487941267521536))/9007199254740992 - (7514214926474921*sin(q3L)*((16506520352940097956833727997725*cos(q2L))/20282409603651670423947251286016 + (7514214926474921*cos(q2L)*((1888752292310023*cos(q1L))/18014398509481984 - 